simulink model "deltino"  (R2021b)
(part 4 of 10)

t2190 = t1608.*t2164;
t2191 = t1609.*t2165;
t2193 = t1606.*t2166;
t2194 = t1607.*t2167;
t2196 = t1632.*t2168;
t2197 = t1633.*t2169;
t2198 = t1630.*t2170;
t2199 = t1631.*t2171;
t2205 = -t2201;
t2206 = -t2202;
t2210 = -t2204;
t2211 = -t2207;
t2213 = -t2208;
t2214 = -t2209;
t2215 = -t2212;
t2216 = t1369+t1722+t1745+t2007;
t2217 = t1371+t1724+t1748+t2008;
t2218 = t1373+t1726+t1751+t2009;
t2219 = t1375+t1728+t1754+t2010;
t2220 = t1370+t1723+t1746+t2022;
t2221 = t1372+t1725+t1749+t2023;
t2222 = t1374+t1727+t1752+t2024;
t2223 = t1376+t1729+t1755+t2025;
t2224 = t1422+t1689+t1758+t2026;
t2225 = t1425+t1692+t1764+t2028;
t2226 = t1428+t1695+t1770+t2030;
t2227 = t1431+t1698+t1776+t2032;
t2228 = t1458+t1660+t1788+t2027;
t2229 = t1459+t1661+t1789+t2029;
t2230 = t1460+t1662+t1791+t2031;
t2231 = t1461+t1663+t1794+t2033;
t2232 = p2x_dot+t47+t454+t459+t472+t480+t482+t643+t699+t872+t893+t910+t1060+t1064+t1076+t1207+t1211+t1317+t1763;
t2233 = p1x_dot+t47+t442+t454+t459+t472+t482+t641+t790+t872+t932+t1048+t1058+t1060+t1064+t1206+t1210+t1314+t1757;
t2234 = p3x_dot+t47+t454+t459+t480+t645+t699+t767+t791+t872+t893+t910+t1060+t1064+t1076+t1208+t1212+t1320+t1769;
t2235 = t1871+t1975+t1996;
t2236 = p4x_dot+t47+t442+t454+t459+t647+t767+t790+t791+t872+t932+t1048+t1058+t1060+t1064+t1209+t1213+t1323+t1775;
t2237 = t1865+t1989+t1997;
t2238 = t1864+t1995+t2001;
t2241 = p2y_dot+t50+t477+t493+t700+t719+t726+t758+t761+t887+t909+t915+t922+t928+t1077+t1215+t1263+t1451+t1735;
t2242 = p3y_dot+t50+t449+t477+t700+t720+t758+t761+t800+t887+t909+t915+t922+t928+t1077+t1216+t1264+t1454+t1738;
t2243 = t1856+t2002+t2006;
t2246 = p1y_dot+t50+t457+t460+t477+t493+t700+t718+t726+t887+t909+t1061+t1067+t1073+t1077+t1214+t1262+t1450+t1732;
t2247 = p4y_dot+t50+t449+t457+t460+t477+t700+t721+t800+t887+t909+t1061+t1067+t1073+t1077+t1217+t1265+t1457+t1741;
t2272 = t1549.*t2248;
t2273 = t1550.*t2249;
t2274 = t1578.*t2252;
t2275 = t1548.*t2253;
t2276 = t1579.*t2256;
t2277 = t1547.*t2257;
t2278 = t1577.*t2258;
t2279 = t1576.*t2259;
t2323 = p2y_dot+t50+t477+t493+t700+t726+t758+t761+t887+t909+t915+t922+t928+t1077+t1453+t1704+t1737+t2067;
t2324 = p3y_dot+t50+t449+t477+t700+t758+t761+t800+t887+t909+t915+t922+t928+t1077+t1456+t1706+t1740+t2069;
t1944 = -t1937;
t1947 = -t1941;
t1966 = p3y+t48+t1949;
t2112 = p3x+t45+t2084;
t2113 = p3x+t45+t2085;
t2114 = p4x+t45+t2086;
t2115 = p4x+t45+t2087;
t2116 = -t2105;
t2117 = p1x+t45+t2088;
t2118 = p1x+t45+t2089;
t2119 = p2x+t45+t2090;
t2120 = p2x+t45+t2091;
t2123 = p3y+t48+t2093;
t2127 = by+t57+t2102;
t2128 = p2y+t48+t2103;
t2132 = by+t59+t2108;
t2134 = p3y+t48+t2111;
t2145 = -t1983.*(t1230-t1555);
t2147 = -t1985.*(t1232-t1557);
t2149 = t1828.*t1994;
t2150 = -t1990.*(t1226-t1551);
t2152 = -t1992.*(t1228-t1553);
t2154 = t1826.*t1999;
t2155 = t1827.*t2000;
t2156 = t1983.*(t1230-t1555);
t2157 = t1829.*t2004;
t2163 = -t2034.*(t1276-t1561);
t2176 = t1919.*t2047;
t2177 = -t2173;
t2178 = t1921.*t2049;
t2179 = t1923.*t2046;
t2180 = -t2175;
t2181 = t1924.*t2048;
t2182 = t1953.*t2016;
t2183 = t1954.*t2017;
t2184 = t1956.*t2014;
t2185 = t1957.*t2015;
t2186 = t1955.*t2018;
t2187 = t1958.*t2021;
t2188 = t1959.*t2019;
t2195 = -t2190;
t2200 = -t2197;
t2239 = 1.0./t2235;
t2244 = 1.0./t2237;
t2250 = 1.0./t2238;
t2254 = 1.0./t2243;
t2260 = t1515.*t2232;
t2261 = t1514.*t2233;
t2263 = t1516.*t2234;
t2265 = t1517.*t2236;
t2268 = -t2241.*(t404-(t7.*t1159)./5.0);
t2269 = -t2242.*(t405-(t10.*t1159)./5.0);
t2270 = -t2246.*(t403-(t4.*t1159)./5.0);
t2271 = -t2247.*(t406-(t13.*t1159)./5.0);
t2280 = t1929+t2109+t2121;
t2281 = t1927+t2110+t2130;
t2282 = t1930+t2106+t2126;
t2301 = t2122.*t2224;
t2306 = t2129.*t2227;
t2310 = t2131.*t2225;
t2315 = p2x_dot+t47+t454+t459+t472+t480+t482+t699+t872+t893+t910+t1060+t1064+t1076+t1318+t1718+t1765+t2073;
t2316 = bx_dot+t65+t472+t480+t482+t699+t755+t760+t893+t910+t914+t918+t1039+t1076+t1365+t1699+t1793+t2056;
t2317 = p1x_dot+t47+t442+t454+t459+t472+t482+t790+t872+t932+t1048+t1058+t1060+t1064+t1315+t1716+t1759+t2072;
t2318 = p2x_dot+t47+t454+t459+t472+t480+t482+t699+t872+t893+t910+t1060+t1064+t1076+t1319+t1719+t1767+t2075;
t2319 = bx_dot+t64+t442+t472+t482+t755+t760+t790+t914+t918+t932+t1039+t1048+t1058+t1363+t1696+t1790+t2055;
t2320 = bx_dot+t65+t472+t480+t482+t699+t755+t760+t893+t910+t914+t918+t1039+t1076+t1366+t1700+t1795+t2063;
t2321 = p1x_dot+t47+t442+t454+t459+t472+t482+t790+t872+t932+t1048+t1058+t1060+t1064+t1316+t1717+t1761+t2074;
t2322 = bx_dot+t64+t442+t472+t482+t755+t760+t790+t914+t918+t932+t1039+t1048+t1058+t1364+t1697+t1792+t2062;
t2325 = by_dot+t71+t443+t449+t758+t761+t788+t800+t915+t922+t928+t933+t1045+t1057+t1410+t1720+t1780+t2064;
t2326 = by_dot+t71+t443+t449+t758+t761+t788+t800+t915+t922+t928+t933+t1045+t1057+t1411+t1665+t1781+t2076;
t2327 = p2y_dot+t50+t477+t493+t700+t726+t758+t761+t887+t909+t915+t922+t928+t1077+t1452+t1703+t1736+t2077;
t2328 = p3y_dot+t50+t449+t477+t700+t758+t761+t800+t887+t909+t915+t922+t928+t1077+t1455+t1705+t1739+t2078;
t2329 = by_dot+t72+t443+t493+t726+t758+t761+t788+t915+t922+t928+t933+t1045+t1057+t1419+t1721+t1782+t2070;
t2330 = by_dot+t72+t443+t493+t726+t758+t761+t788+t915+t922+t928+t933+t1045+t1057+t1420+t1668+t1783+t2079;
t2336 = -1.0./(-t1932+t1985.*(t1232-t1557)+t2003.*(t1281-t1562));
t2337 = 1.0./(-t1932+t1985.*(t1232-t1557)+t2003.*(t1281-t1562)).^2;
t2343 = -1.0./(t1933+t1990.*(t1226-t1551)+t1998.*(t1266-t1559));
t2344 = 1.0./(t1933+t1990.*(t1226-t1551)+t1998.*(t1266-t1559)).^2;
t2351 = -1.0./(t1931+t1992.*(t1228-t1553)+t2011.*(t1271-t1560));
t2352 = 1.0./(t1931+t1992.*(t1228-t1553)+t2011.*(t1271-t1560)).^2;
t2364 = t1889.*t2323;
t2365 = t1890.*t2324;
t2380 = (t2165.*-2.0e+2)./(-t1932+t1985.*(t1232-t1557)+t2003.*(t1281-t1562));
t2381 = (t2165.*2.0e+2)./(-t1932+t1985.*(t1232-t1557)+t2003.*(t1281-t1562));
t2383 = (t2166.*-2.0e+2)./(t1933+t1990.*(t1226-t1551)+t1998.*(t1266-t1559));
t2386 = (t2166.*2.0e+2)./(t1933+t1990.*(t1226-t1551)+t1998.*(t1266-t1559));
t2387 = (t2167.*-2.0e+2)./(t1931+t1992.*(t1228-t1553)+t2011.*(t1271-t1560));
t2392 = (t2167.*2.0e+2)./(t1931+t1992.*(t1228-t1553)+t2011.*(t1271-t1560));
t2436 = t2036+t2124+t2203+t2205+t2272+t2274;
t2437 = t2038+t2125+t2206+t2210+t2273+t2276;
t2438 = t2037+t2136+t2214+t2215+t2275+t2278;
t2439 = t2039+t2135+t2211+t2213+t2277+t2279;
t2133 = -t1966.*(t405-(t10.*t1159)./5.0);
t2160 = -t2157;
t2189 = t1966.*t2020;
t2240 = t2239.^2;
t2245 = t2244.^2;
t2251 = t2250.^2;
t2255 = t2254.^2;
t2262 = -t2260;
t2264 = -t2261;
t2266 = -t2263;
t2267 = -t2265;
t2284 = 1.0./t2280;
t2286 = 1.0./t2281;
t2288 = 1.0./t2282;
t2290 = -1.0./(t2105+t1853.*(t211./5.0-t248)+t1966.*(t405-(t10.*t1159)./5.0));
t2291 = 1.0./(t2105+t1853.*(t211./5.0-t248)+t1966.*(t405-(t10.*t1159)./5.0)).^2;
t2292 = t2112.*t2218;
t2293 = t2114.*t2219;
t2294 = t2117.*t2216;
t2295 = t2119.*t2217;
t2296 = t2113.*t2222;
t2297 = t2115.*t2223;
t2298 = t2118.*t2220;
t2299 = t2120.*t2221;
t2305 = t2123.*t2230;
t2309 = t2127.*t2228;
t2311 = t2128.*t2229;
t2312 = t2134.*t2226;
t2313 = t2132.*t2231;
t2331 = t1932+t2147+t2161;
t2332 = t1947+t2146+t2149;
t2333 = t1936+t2150+t2159;
t2334 = t1944+t2153+t2155;
t2338 = t1940+t2154+t2158;
t2339 = t1935+t2152+t2162;
t2340 = t1934+t2156+t2163;
t2341 = -1.0./(t1941-t2149+t1984.*(t1231-t1556));
t2342 = 1.0./(t1941-t2149+t1984.*(t1231-t1556)).^2;
t2345 = -1.0./(t1937-t2155+t1993.*(t1229-t1554));
t2346 = 1.0./(t1937-t2155+t1993.*(t1229-t1554)).^2;
t2347 = -1.0./(-t1938+t2157+t1986.*(t1233-t1558));
t2348 = 1.0./(-t1938+t2157+t1986.*(t1233-t1558)).^2;
t2355 = t2315.*(t1679-(t8.*t1070)./5.0);
t2356 = t2316.*(t1683-(t14.*t1070)./5.0);
t2357 = t2317.*(t1677-(t5.*t1070)./5.0);
t2358 = t2318.*(t1680-(t9.*t1070)./5.0);
t2359 = t2319.*(t1681-(t11.*t1070)./5.0);
t2360 = t2320.*(t1684-(t15.*t1070)./5.0);
t2361 = t2321.*(t1678-(t6.*t1070)./5.0);
t2362 = t2322.*(t1682-(t12.*t1070)./5.0);
t2367 = t1888.*t2326;
t2368 = t1891.*t2330;
t2369 = t2325.*(t1685-(t5.*t1159)./5.0);
t2371 = t2327.*(t1686-(t8.*t1159)./5.0);
t2372 = t2328.*(t1687-(t11.*t1159)./5.0);
t2373 = t2329.*(t1688-(t14.*t1159)./5.0);
t2379 = t2080./(t2105+t1853.*(t211./5.0-t248)+t1966.*(t405-(t10.*t1159)./5.0));
t2382 = (t2168.*-2.0e+2)./(t1941-t2149+t1984.*(t1231-t1556));
t2384 = (t2168.*2.0e+2)./(t1941-t2149+t1984.*(t1231-t1556));
t2385 = (t2169.*-2.0e+2)./(-t1938+t2157+t1986.*(t1233-t1558));
t2388 = (t2171.*-2.0e+2)./(t1937-t2155+t1993.*(t1229-t1554));
t2390 = (t2169.*2.0e+2)./(-t1938+t2157+t1986.*(t1233-t1558));
t2393 = (t2171.*2.0e+2)./(t1937-t2155+t1993.*(t1229-t1554));
t2408 = (t2316.*-2.0e+2)./(-t1932+t1985.*(t1232-t1557)+t2003.*(t1281-t1562));
t2409 = (t2316.*2.0e+2)./(-t1932+t1985.*(t1232-t1557)+t2003.*(t1281-t1562));
t2410 = (t2324.*-2.0e+2)./(t1941-t2149+t1984.*(t1231-t1556));
t2411 = (t2329.*-2.0e+2)./(-t1932+t1985.*(t1232-t1557)+t2003.*(t1281-t1562));
t2412 = (t2317.*-2.0e+2)./(t1933+t1990.*(t1226-t1551)+t1998.*(t1266-t1559));
t2413 = (t2315.*-2.0e+2)./(t1931+t1992.*(t1228-t1553)+t2011.*(t1271-t1560));
t2414 = (t2318.*-2.0e+2)./(t1937-t2155+t1993.*(t1229-t1554));
t2415 = (t2322.*-2.0e+2)./(t1941-t2149+t1984.*(t1231-t1556));
t2416 = (t2320.*-2.0e+2)./(-t1938+t2157+t1986.*(t1233-t1558));
t2417 = (t2323.*-2.0e+2)./(t1937-t2155+t1993.*(t1229-t1554));
t2418 = (t2329.*2.0e+2)./(-t1932+t1985.*(t1232-t1557)+t2003.*(t1281-t1562));
t2419 = (t2322.*2.0e+2)./(t1941-t2149+t1984.*(t1231-t1556));
t2420 = (t2320.*2.0e+2)./(-t1938+t2157+t1986.*(t1233-t1558));
t2423 = (t2325.*-2.0e+2)./(t1933+t1990.*(t1226-t1551)+t1998.*(t1266-t1559));
t2424 = (t2330.*-2.0e+2)./(-t1938+t2157+t1986.*(t1233-t1558));
t2426 = (t2325.*2.0e+2)./(t1933+t1990.*(t1226-t1551)+t1998.*(t1266-t1559));
t2428 = (t2327.*-2.0e+2)./(t1931+t1992.*(t1228-t1553)+t2011.*(t1271-t1560));
t2429 = (t2330.*2.0e+2)./(-t1938+t2157+t1986.*(t1233-t1558));
t2192 = -t2189;
t2283 = t1926+t2116+t2133;
t2285 = t2284.^2;
t2287 = t2286.^2;
t2289 = t2288.^2;
t2300 = -t2293;
t2302 = -t2294;
t2303 = -t2295;
t2304 = -t2296;
t2307 = -t2298;
t2308 = -t2299;
t2314 = -t2309;
t2335 = t1938+t2148+t2160;
t2349 = 1.0./t2338;
t2353 = 1.0./t2340;
t2363 = -t2356;
t2366 = -t2362;
t2370 = -t2367;
t2374 = -t2371;
t2375 = t2082.*t2284;
t2376 = t2081.*t2288;
t2377 = t2083.*t2286;
t2378 = t2080.*t2290;
t2394 = t2233.*t2284;
t2395 = t2232.*t2286;
t2398 = t2234.*t2290;
t2399 = t2236.*t2288;
t2401 = t2246.*t2284;
t2402 = t2241.*t2286;
t2403 = t2242.*t2290;
t2404 = t2247.*t2288;
t2432 = t2050+t2144+t2185+t2188+t2262+t2268;
t2433 = t2051+t2143+t2184+t2186+t2264+t2270;
t2434 = t2057+t2142+t2183+t2187+t2267+t2271;
t2465 = t2180+t2195+t2292+t2312+t2359+t2372;
t2467 = t2178+t2200+t2297+t2313+t2360+t2368;
t2481 = t1916.*t2337.*(t2173-t2191+t2293-t2306+t2356-t2373).*-4.0e+4;
t2495 = t2114.*t2337.*(t2173-t2191+t2293-t2306+t2356-t2373).*-4.0e+4;
t2496 = t2114.*t2337.*(t2173-t2191+t2293-t2306+t2356-t2373).*4.0e+4;
t2498 = t2129.*t2337.*(t2173-t2191+t2293-t2306+t2356-t2373).*-4.0e+4;
t2350 = t2349.^2;
t2354 = t2353.^2;
t2389 = t2164.*t2353.*2.0e+2;
t2391 = t2170.*t2349.*2.0e+2;
t2396 = -t2394;
t2397 = -t2395;
t2400 = -t2399;
t2405 = -t2401;
t2406 = -t2402;
t2407 = -t2404;
t2421 = t2321.*t2349.*2.0e+2;
t2422 = t2319.*t2353.*2.0e+2;
t2427 = t2326.*t2349.*2.0e+2;
t2430 = t2328.*t2353.*2.0e+2;
t2435 = t2052+t2141+t2182+t2192+t2266+t2269;
t2440 = t1848.*t2287.*t2432;
t2441 = t1852.*t2285.*t2433;
t2444 = t1861.*t2289.*t2434;
t2448 = t1955.*t2285.*t2433;
t2449 = t1956.*t2285.*t2433;
t2450 = t1957.*t2287.*t2432;
t2451 = t1959.*t2287.*t2432;
t2454 = t1954.*t2289.*t2434;
t2455 = t1958.*t2289.*t2434;
t2461 = t2174+t2193+t2301+t2302+t2357+t2369;
t2462 = t2177+t2191+t2300+t2306+t2363+t2373;
t2463 = t2172+t2194+t2303+t2310+t2355+t2374;
t2464 = t2176+t2199+t2308+t2311+t2358+t2364;
t2466 = t2181+t2196+t2304+t2305+t2365+t2366;
t2468 = t2179+t2198+t2307+t2314+t2361+t2370;
t2489 = t1921.*t2348.*t2467.*4.0e+4;
t2504 = t2115.*t2348.*t2467.*4.0e+4;
t2514 = t2132.*t2348.*t2467.*4.0e+4;
t2520 = t2381+t2481;
t2528 = t2409+t2496;
t2530 = t2418+t2498;
t2425 = -t2421;
t2431 = -t2430;
t2442 = -t2440;
t2443 = -t2441;
t2445 = t1853.*t2291.*t2435;
t2446 = -t2444;
t2447 = (t1853.*t2290.*t2435)./(t2105+t1853.*(t211./5.0-t248)+t1966.*(t405-(t10.*t1159)./5.0));
t2452 = -t2449;
t2453 = -t2450;
t2456 = t1953.*t2291.*t2435;
t2457 = -t2454;
t2458 = (t1953.*t2290.*t2435)./(t2105+t1853.*(t211./5.0-t248)+t1966.*(t405-(t10.*t1159)./5.0));
t2459 = t1966.*t2291.*t2435;
t2460 = (t1966.*t2290.*t2435)./(t2105+t1853.*(t211./5.0-t248)+t1966.*(t405-(t10.*t1159)./5.0));
t2475 = t2405+t2448;
t2476 = t2406+t2451;
t2479 = t2407+t2455;
t2482 = t1918.*t2344.*t2461.*4.0e+4;
t2484 = t1915.*t2352.*t2463.*4.0e+4;
t2485 = t1919.*t2346.*t2464.*4.0e+4;
t2488 = t1924.*t2342.*t2466.*4.0e+4;
t2491 = -t2489;
t2492 = t1920.*t2354.*t2465.*4.0e+4;
t2493 = t1923.*t2350.*t2468.*4.0e+4;
t2497 = t2117.*t2344.*t2461.*4.0e+4;
t2500 = t2113.*t2342.*t2466.*4.0e+4;
t2501 = t2122.*t2344.*t2461.*4.0e+4;
t2502 = t2120.*t2346.*t2464.*4.0e+4;
t2505 = t2119.*t2352.*t2463.*4.0e+4;
t2507 = t2123.*t2342.*t2466.*4.0e+4;
t2509 = t2112.*t2354.*t2465.*4.0e+4;
t2510 = t2128.*t2346.*t2464.*4.0e+4;
t2513 = t2131.*t2352.*t2463.*4.0e+4;
t2515 = -t2514;
t2516 = t2134.*t2354.*t2465.*4.0e+4;
t2517 = t2118.*t2350.*t2468.*4.0e+4;
t2519 = t2127.*t2350.*t2468.*4.0e+4;
S_dot = ft_5({bx,bx_dot,by,by_dot,p1x,p1x_dot,p1y,p1y_dot,p2x,p2x_dot,p2y,p2y_dot,p4x,p4x_dot,p4y,p4y_dot,phi_dot,psi_dot,t10,t1006,t1012,t1013,t1014,t1015,t1016,t1018,t102,t1027,t1028,t1030,t1031,t1033,t1037,t1039,t1040,t1045,t1046,t1047,t1048,t1049,t1051,t1052,t1053,t1054,t1056,t1057,t1058,t1059,t1060,t1061,t1062,t1063,t1064,t1065,t1066,t1067,t1069,t1070,t1071,t1072,t1073,t1074,t1075,t1076,t1077,t1078,t1079,t1081,t1083,t1084,t1086,t1087,t1089,t1091,t1092,t1093,t1094,t1096,t1098,t11,t1105,t1106,t1108,t1109,t1111,t1115,t1126,t1127,t1129,t1131,t1133,t1134,t1135,t1136,t1138,t1139,t1150,t1151,t1159,t1160,t1165,t1171,t1172,t12,t1208,t1212,t1216,t1226,t1228,t1229,t1231,t1232,t1233,t1264,t1266,t1271,t1281,t13,t1315,t1316,t1318,t1319,t1320,t1326,t1365,t1366,t1367,t1393,t14,t1408,t1410,t1411,t1436,t144,t145,t1452,t1453,t1454,t1455,t1456,t146,t147,t148,t149,t15,t150,t151,t152,t153,t1533,t1534,t154,t155,t1551,t1553,t1554,t1556,t1557,t1558,t1559,t1560,t1562,t1564,t1570,t1571,t1572,t1582,t1583,t1599,t16,t1600,t1601,t161,t1610,t1611,t1614,t162,t1629,t163,t1634,t1635,t1636,t1637,t164,t1642,t1643,t1644,t1645,t165,t166,t1664,t1665,t1699,t17,t1700,t1701,t1703,t1704,t1705,t1706,t1707,t1716,t1717,t1718,t1719,t1720,t1730,t1731,t1736,t1737,t1738,t1739,t1740,t1742,t1743,t175,t1759,t176,t1761,t1765,t1767,t1769,t177,t1771,t1773,t1780,t1781,t1793,t1795,t1796,t18,t180,t1809,t181,t1810,t1823,t183,t1847,t1851,t1853,t1858,t1859,t1860,t1866,t1867,t1868,t187,t1872,t1873,t1874,t1875,t1876,t1877,t1878,t1879,t1896,t1897,t1898,t1899,t19,t190,t1900,t1901,t1902,t1903,t1904,t1905,t1906,t1907,t1915,t1916,t1918,t1919,t1920,t1921,t1923,t1924,t1931,t1932,t1933,t1937,t1938,t1939,t1941,t1942,t1943,t1945,t1946,t1948,t1949,t1950,t1951,t1952,t1953,t1960,t1961,t1962,t1963,t1964,t1965,t1966,t1967,t1968,t1969,t1970,t1971,t1972,t1973,t1974,t1984,t1985,t1986,t1990,t1992,t1993,t1998,t2,t20,t2003,t2005,t2011,t2012,t2013,t2035,t2044,t2045,t2055,t2056,t2058,t2059,t2062,t2063,t2064,t2067,t2069,t207,t2070,t2071,t2072,t2073,t2074,t2075,t2076,t2077,t2078,t208,t2084,t2085,t2086,t2087,t2088,t2089,t209,t2090,t2091,t2092,t2093,t21,t210,t2102,t2103,t2104,t2105,t2107,t2108,t211,t2111,t2112,t2113,t2114,t2115,t2117,t2118,t2119,t212,t2120,t2122,t2123,t2127,t2128,t2129,t2131,t2132,t2134,t214,t2149,t2155,t2157,t2164,t2165,t2166,t2167,t2168,t2169,t217,t2170,t2171,t2173,t218,t219,t2191,t22,t2201,t2202,t2203,t2204,t2207,t2208,t2209,t221,t2212,t222,t223,t2234,t2239,t2240,t2242,t2244,t2245,t2248,t2249,t225,t2250,t2251,t2252,t2253,t2254,t2255,t2256,t2257,t2258,t2259,t2272,t2273,t2274,t2275,t2276,t2277,t2278,t2279,t2290,t2293,t23,t2306,t2315,t2316,t2317,t2318,t2319,t2320,t2321,t2322,t2323,t2324,t2325,t2326,t2327,t2328,t2329,t233,t2330,t2337,t2342,t2344,t2346,t2348,t2349,t2350,t2352,t2353,t2354,t2356,t236,t237,t2373,t2375,t2376,t2377,t2379,t238,t2384,t2386,t2389,t2390,t2391,t2392,t2393,t2396,t2397,t2398,t24,t2400,t2403,t241,t2410,t2412,t2413,t2414,t2417,t2419,t242,t2420,t2422,t2425,t2426,t2427,t2428,t2429,t243,t2431,t2435,t244,t2442,t2443,t2446,t2447,t245,t2452,t2453,t2457,t2458,t246,t2460,t2461,t2463,t2464,t2465,t2466,t2467,t2468,t247,t2475,t2476,t2479,t248,t2482,t2484,t2485,t2488,t249,t2491,t2492,t2493,t2497,t25,t2500,t2501,t2502,t2504,t2505,t2507,t2509,t2510,t2513,t2515,t2516,t2517,t2519,t252,t2520,t2528,t2530,t254,t255,t256,t257,t258,t26,t260,t261,t265,t267,t27,t270,t272,t273,t28,t29,t3,t30,t308,t31,t312,t316,t317,t318,t319,t322,t324,t328,t329,t341,t343,t350,t351,t352,t353,t354,t358,t359,t360,t361,t362,t366,t367,t368,t369,t371,t374,t375,t376,t377,t379,t380,t381,t383,t4,t402,t403,t404,t405,t406,t419,t420,t422,t423,t424,t427,t429,t431,t437,t442,t443,t444,t445,t446,t449,t450,t454,t455,t456,t457,t458,t459,t460,t461,t462,t464,t465,t470,t471,t472,t474,t475,t477,t478,t479,t480,t481,t482,t483,t485,t486,t488,t489,t490,t492,t493,t494,t5,t501,t502,t504,t529,t530,t531,t532,t533,t535,t536,t539,t540,t541,t542,t543,t544,t545,t548,t549,t552,t558,t561,t562,t563,t570,t572,t577,t578,t580,t6,t601,t603,t607,t609,t610,t612,t614,t620,t641,t643,t645,t647,t661,t663,t667,t669,t670,t672,t673,t674,t676,t678,t680,t684,t698,t699,t7,t700,t701,t718,t719,t720,t721,t722,t723,t725,t726,t728,t731,t733,t737,t754,t755,t756,t757,t758,t759,t760,t761,t762,t763,t765,t767,t768,t77,t770,t771,t777,t778,t78,t780,t781,t783,t784,t786,t787,t788,t789,t79,t790,t791,t792,t794,t795,t796,t797,t798,t799,t8,t80,t800,t801,t802,t804,t805,t806,t807,t808,t809,t81,t814,t815,t816,t817,t82,t825,t827,t831,t836,t837,t84,t840,t845,t846,t847,t848,t85,t851,t86,t87,t872,t873,t88,t882,t885,t887,t888,t889,t89,t890,t891,t892,t893,t894,t896,t9,t90,t907,t908,t909,t91,t910,t911,t913,t914,t915,t916,t917,t918,t919,t92,t920,t921,t922,t924,t925,t926,t927,t928,t93,t930,t932,t933,t934,t935,t936,t94,t945,t947,t949,t95,t951,t953,t954,t955,t957,t959,t961,t963,t964,t966,t967,t972,t981,t982,t984,t985,t987,t991,t993,t995,t999,th11_dot,th12_dot,th13_dot,th21_dot,th22_dot,th23_dot,th31_dot,th32_dot,th33_dot,th41_dot,th42_dot,th43_dot,zeta_dot});
end
function S_dot = ft_5(ct)
bx = ct{1};
bx_dot = ct{2};
by = ct{3};
by_dot = ct{4};
p1x = ct{5};
p1x_dot = ct{6};
p1y = ct{7};
p1y_dot = ct{8};
p2x = ct{9};
p2x_dot = ct{10};
p2y = ct{11};
p2y_dot = ct{12};
p4x = ct{13};
p4x_dot = ct{14};
p4y = ct{15};
p4y_dot = ct{16};
phi_dot = ct{17};
psi_dot = ct{18};
t10 = ct{19};
t1006 = ct{20};
t1012 = ct{21};
t1013 = ct{22};
t1014 = ct{23};
t1015 = ct{24};
t1016 = ct{25};
t1018 = ct{26};
t102 = ct{27};
t1027 = ct{28};
t1028 = ct{29};
t1030 = ct{30};
t1031 = ct{31};
t1033 = ct{32};
t1037 = ct{33};
t1039 = ct{34};
t1040 = ct{35};
t1045 = ct{36};
t1046 = ct{37};
t1047 = ct{38};
t1048 = ct{39};
t1049 = ct{40};
t1051 = ct{41};
t1052 = ct{42};
t1053 = ct{43};
t1054 = ct{44};
t1056 = ct{45};
t1057 = ct{46};
t1058 = ct{47};
t1059 = ct{48};
t1060 = ct{49};
t1061 = ct{50};
t1062 = ct{51};
t1063 = ct{52};
t1064 = ct{53};
t1065 = ct{54};
t1066 = ct{55};
t1067 = ct{56};
t1069 = ct{57};
t1070 = ct{58};
t1071 = ct{59};
t1072 = ct{60};
t1073 = ct{61};
t1074 = ct{62};
t1075 = ct{63};
t1076 = ct{64};
t1077 = ct{65};
t1078 = ct{66};
t1079 = ct{67};
t1081 = ct{68};
t1083 = ct{69};
t1084 = ct{70};
t1086 = ct{71};
t1087 = ct{72};
t1089 = ct{73};
t1091 = ct{74};
t1092 = ct{75};
t1093 = ct{76};
t1094 = ct{77};
t1096 = ct{78};
t1098 = ct{79};
t11 = ct{80};
t1105 = ct{81};
t1106 = ct{82};
t1108 = ct{83};
t1109 = ct{84};
t1111 = ct{85};
t1115 = ct{86};
t1126 = ct{87};
t1127 = ct{88};
t1129 = ct{89};
t1131 = ct{90};
t1133 = ct{91};
t1134 = ct{92};
t1135 = ct{93};
t1136 = ct{94};
t1138 = ct{95};
t1139 = ct{96};
t1150 = ct{97};
t1151 = ct{98};
t1159 = ct{99};
t1160 = ct{100};
t1165 = ct{101};
t1171 = ct{102};
t1172 = ct{103};
t12 = ct{104};
t1208 = ct{105};
t1212 = ct{106};
t1216 = ct{107};
t1226 = ct{108};
t1228 = ct{109};
t1229 = ct{110};
t1231 = ct{111};
t1232 = ct{112};
t1233 = ct{113};
t1264 = ct{114};
t1266 = ct{115};
t1271 = ct{116};
t1281 = ct{117};
t13 = ct{118};
t1315 = ct{119};
t1316 = ct{120};
t1318 = ct{121};
t1319 = ct{122};
t1320 = ct{123};
t1326 = ct{124};
t1365 = ct{125};
t1366 = ct{126};
t1367 = ct{127};
t1393 = ct{128};
t14 = ct{129};
t1408 = ct{130};
t1410 = ct{131};
t1411 = ct{132};
t1436 = ct{133};
t144 = ct{134};
t145 = ct{135};
t1452 = ct{136};
t1453 = ct{137};
t1454 = ct{138};
t1455 = ct{139};
t1456 = ct{140};
t146 = ct{141};
t147 = ct{142};
t148 = ct{143};
t149 = ct{144};
t15 = ct{145};
t150 = ct{146};
t151 = ct{147};
t152 = ct{148};
t153 = ct{149};
t1533 = ct{150};
t1534 = ct{151};
t154 = ct{152};
t155 = ct{153};
t1551 = ct{154};
t1553 = ct{155};
t1554 = ct{156};
t1556 = ct{157};
t1557 = ct{158};
t1558 = ct{159};
t1559 = ct{160};
t1560 = ct{161};
t1562 = ct{162};
t1564 = ct{163};
t1570 = ct{164};
t1571 = ct{165};
t1572 = ct{166};
t1582 = ct{167};
t1583 = ct{168};
t1599 = ct{169};
t16 = ct{170};
t1600 = ct{171};
t1601 = ct{172};
t161 = ct{173};
t1610 = ct{174};
t1611 = ct{175};
t1614 = ct{176};
t162 = ct{177};
t1629 = ct{178};
t163 = ct{179};
t1634 = ct{180};
t1635 = ct{181};
t1636 = ct{182};
t1637 = ct{183};
t164 = ct{184};
t1642 = ct{185};
t1643 = ct{186};
t1644 = ct{187};
t1645 = ct{188};
t165 = ct{189};
t166 = ct{190};
t1664 = ct{191};
t1665 = ct{192};
t1699 = ct{193};
t17 = ct{194};
t1700 = ct{195};
t1701 = ct{196};
t1703 = ct{197};
t1704 = ct{198};
t1705 = ct{199};
t1706 = ct{200};
t1707 = ct{201};
t1716 = ct{202};
t1717 = ct{203};
t1718 = ct{204};
t1719 = ct{205};
t1720 = ct{206};
t1730 = ct{207};
t1731 = ct{208};
t1736 = ct{209};
t1737 = ct{210};
t1738 = ct{211};
t1739 = ct{212};
t1740 = ct{213};
t1742 = ct{214};
t1743 = ct{215};
t175 = ct{216};
t1759 = ct{217};
t176 = ct{218};
t1761 = ct{219};
t1765 = ct{220};
t1767 = ct{221};
t1769 = ct{222};
t177 = ct{223};
t1771 = ct{224};
t1773 = ct{225};
t1780 = ct{226};
t1781 = ct{227};
t1793 = ct{228};
t1795 = ct{229};
t1796 = ct{230};
t18 = ct{231};
t180 = ct{232};
t1809 = ct{233};
t181 = ct{234};
t1810 = ct{235};
t1823 = ct{236};
t183 = ct{237};
t1847 = ct{238};
t1851 = ct{239};
t1853 = ct{240};
t1858 = ct{241};
t1859 = ct{242};
t1860 = ct{243};
t1866 = ct{244};
t1867 = ct{245};
t1868 = ct{246};
t187 = ct{247};
t1872 = ct{248};
t1873 = ct{249};
t1874 = ct{250};
t1875 = ct{251};
t1876 = ct{252};
t1877 = ct{253};
t1878 = ct{254};
t1879 = ct{255};
t1896 = ct{256};
t1897 = ct{257};
t1898 = ct{258};
t1899 = ct{259};
t19 = ct{260};
t190 = ct{261};
t1900 = ct{262};
t1901 = ct{263};
t1902 = ct{264};
t1903 = ct{265};
t1904 = ct{266};
t1905 = ct{267};
t1906 = ct{268};
t1907 = ct{269};
t1915 = ct{270};
t1916 = ct{271};
t1918 = ct{272};
t1919 = ct{273};
t1920 = ct{274};
t1921 = ct{275};
t1923 = ct{276};
t1924 = ct{277};
t1931 = ct{278};
t1932 = ct{279};
t1933 = ct{280};
t1937 = ct{281};
t1938 = ct{282};
t1939 = ct{283};
t1941 = ct{284};
t1942 = ct{285};
t1943 = ct{286};
t1945 = ct{287};
t1946 = ct{288};
t1948 = ct{289};
t1949 = ct{290};
t1950 = ct{291};
t1951 = ct{292};
t1952 = ct{293};
t1953 = ct{294};
t1960 = ct{295};
t1961 = ct{296};
t1962 = ct{297};
t1963 = ct{298};
t1964 = ct{299};
t1965 = ct{300};
t1966 = ct{301};
t1967 = ct{302};
t1968 = ct{303};
t1969 = ct{304};
t1970 = ct{305};
t1971 = ct{306};
t1972 = ct{307};
t1973 = ct{308};
t1974 = ct{309};
t1984 = ct{310};
t1985 = ct{311};
t1986 = ct{312};
t1990 = ct{313};
t1992 = ct{314};
t1993 = ct{315};
t1998 = ct{316};
t2 = ct{317};
t20 = ct{318};
t2003 = ct{319};
t2005 = ct{320};
t2011 = ct{321};
t2012 = ct{322};
t2013 = ct{323};
t2035 = ct{324};
t2044 = ct{325};
t2045 = ct{326};
t2055 = ct{327};
t2056 = ct{328};
t2058 = ct{329};
t2059 = ct{330};
t2062 = ct{331};
t2063 = ct{332};
t2064 = ct{333};
t2067 = ct{334};
t2069 = ct{335};
t207 = ct{336};
t2070 = ct{337};
t2071 = ct{338};
t2072 = ct{339};
t2073 = ct{340};
t2074 = ct{341};
t2075 = ct{342};
t2076 = ct{343};
t2077 = ct{344};
t2078 = ct{345};
t208 = ct{346};
t2084 = ct{347};
t2085 = ct{348};
t2086 = ct{349};
t2087 = ct{350};
t2088 = ct{351};
t2089 = ct{352};
t209 = ct{353};
t2090 = ct{354};
t2091 = ct{355};
t2092 = ct{356};
t2093 = ct{357};
t21 = ct{358};
t210 = ct{359};
t2102 = ct{360};
t2103 = ct{361};
t2104 = ct{362};
t2105 = ct{363};
t2107 = ct{364};
t2108 = ct{365};
t211 = ct{366};
t2111 = ct{367};
t2112 = ct{368};
t2113 = ct{369};
t2114 = ct{370};
t2115 = ct{371};
t2117 = ct{372};
t2118 = ct{373};
t2119 = ct{374};
t212 = ct{375};
t2120 = ct{376};
t2122 = ct{377};
t2123 = ct{378};
t2127 = ct{379};
t2128 = ct{380};
t2129 = ct{381};
t2131 = ct{382};
t2132 = ct{383};
t2134 = ct{384};
t214 = ct{385};
t2149 = ct{386};
t2155 = ct{387};
t2157 = ct{388};
t2164 = ct{389};
t2165 = ct{390};
t2166 = ct{391};
t2167 = ct{392};
t2168 = ct{393};
t2169 = ct{394};
t217 = ct{395};
t2170 = ct{396};
t2171 = ct{397};
t2173 = ct{398};
t218 = ct{399};
t219 = ct{400};
t2191 = ct{401};
t22 = ct{402};
t2201 = ct{403};
t2202 = ct{404};
t2203 = ct{405};
t2204 = ct{406};
t2207 = ct{407};
t2208 = ct{408};
t2209 = ct{409};
t221 = ct{410};
t2212 = ct{411};
t222 = ct{412};
t223 = ct{413};
t2234 = ct{414};
t2239 = ct{415};
t2240 = ct{416};
t2242 = ct{417};
t2244 = ct{418};
t2245 = ct{419};
t2248 = ct{420};
t2249 = ct{421};
t225 = ct{422};
t2250 = ct{423};
t2251 = ct{424};
t2252 = ct{425};
t2253 = ct{426};
t2254 = ct{427};
t2255 = ct{428};
t2256 = ct{429};
t2257 = ct{430};
t2258 = ct{431};
t2259 = ct{432};
t2272 = ct{433};
t2273 = ct{434};
t2274 = ct{435};
t2275 = ct{436};
t2276 = ct{437};
t2277 = ct{438};
t2278 = ct{439};
t2279 = ct{440};
t2290 = ct{441};
t2293 = ct{442};
t23 = ct{443};
t2306 = ct{444};
t2315 = ct{445};
t2316 = ct{446};
t2317 = ct{447};
t2318 = ct{448};
t2319 = ct{449};
t2320 = ct{450};
t2321 = ct{451};
t2322 = ct{452};
t2323 = ct{453};
t2324 = ct{454};
t2325 = ct{455};
t2326 = ct{456};
t2327 = ct{457};
t2328 = ct{458};
t2329 = ct{459};
t233 = ct{460};
t2330 = ct{461};
t2337 = ct{462};
t2342 = ct{463};
t2344 = ct{464};
t2346 = ct{465};
t2348 = ct{466};
t2349 = ct{467};
t2350 = ct{468};
t2352 = ct{469};
t2353 = ct{470};
t2354 = ct{471};
t2356 = ct{472};
t236 = ct{473};
t237 = ct{474};
t2373 = ct{475};
t2375 = ct{476};
t2376 = ct{477};
t2377 = ct{478};
t2379 = ct{479};
t238 = ct{480};
t2384 = ct{481};
t2386 = ct{482};
t2389 = ct{483};
t2390 = ct{484};
t2391 = ct{485};
t2392 = ct{486};
t2393 = ct{487};
t2396 = ct{488};
t2397 = ct{489};
t2398 = ct{490};
t24 = ct{491};
t2400 = ct{492};
t2403 = ct{493};
t241 = ct{494};
t2410 = ct{495};
t2412 = ct{496};
t2413 = ct{497};
t2414 = ct{498};
t2417 = ct{499};
t2419 = ct{500};
t242 = ct{501};
t2420 = ct{502};
t2422 = ct{503};
t2425 = ct{504};
t2426 = ct{505};
t2427 = ct{506};
t2428 = ct{507};
t2429 = ct{508};
t243 = ct{509};
t2431 = ct{510};
t2435 = ct{511};
t244 = ct{512};
t2442 = ct{513};
t2443 = ct{514};
t2446 = ct{515};
t2447 = ct{516};
t245 = ct{517};
t2452 = ct{518};
t2453 = ct{519};
t2457 = ct{520};
t2458 = ct{521};
t246 = ct{522};
t2460 = ct{523};
t2461 = ct{524};
t2463 = ct{525};
t2464 = ct{526};
t2465 = ct{527};
t2466 = ct{528};
t2467 = ct{529};
t2468 = ct{530};
t247 = ct{531};
t2475 = ct{532};
t2476 = ct{533};
t2479 = ct{534};
t248 = ct{535};
t2482 = ct{536};
t2484 = ct{537};
t2485 = ct{538};
t2488 = ct{539};
t249 = ct{540};
t2491 = ct{541};
t2492 = ct{542};
t2493 = ct{543};
t2497 = ct{544};
t25 = ct{545};
t2500 = ct{546};
t2501 = ct{547};
t2502 = ct{548};
t2504 = ct{549};
t2505 = ct{550};
t2507 = ct{551};
t2509 = ct{552};
t2510 = ct{553};
t2513 = ct{554};
t2515 = ct{555};
t2516 = ct{556};
t2517 = ct{557};
t2519 = ct{558};
t252 = ct{559};
t2520 = ct{560};
t2528 = ct{561};
t2530 = ct{562};
t254 = ct{563};
t255 = ct{564};
t256 = ct{565};
t257 = ct{566};
t258 = ct{567};
t26 = ct{568};
t260 = ct{569};
t261 = ct{570};
t265 = ct{571};
t267 = ct{572};
t27 = ct{573};
t270 = ct{574};
t272 = ct{575};
t273 = ct{576};
t28 = ct{577};
t29 = ct{578};
t3 = ct{579};
t30 = ct{580};
t308 = ct{581};
t31 = ct{582};
t312 = ct{583};
t316 = ct{584};
t317 = ct{585};
t318 = ct{586};
t319 = ct{587};
t322 = ct{588};
t324 = ct{589};
t328 = ct{590};
t329 = ct{591};
t341 = ct{592};
t343 = ct{593};
t350 = ct{594};
t351 = ct{595};
t352 = ct{596};
t353 = ct{597};
t354 = ct{598};
t358 = ct{599};
t359 = ct{600};
t360 = ct{601};
t361 = ct{602};
t362 = ct{603};
t366 = ct{604};
t367 = ct{605};
t368 = ct{606};
t369 = ct{607};
t371 = ct{608};
t374 = ct{609};
t375 = ct{610};
t376 = ct{611};
t377 = ct{612};
t379 = ct{613};
t380 = ct{614};
t381 = ct{615};
t383 = ct{616};
t4 = ct{617};
t402 = ct{618};
t403 = ct{619};
t404 = ct{620};
t405 = ct{621};
t406 = ct{622};
t419 = ct{623};
t420 = ct{624};
t422 = ct{625};
t423 = ct{626};
t424 = ct{627};
t427 = ct{628};
t429 = ct{629};
t431 = ct{630};
t437 = ct{631};
t442 = ct{632};
t443 = ct{633};
t444 = ct{634};
t445 = ct{635};
t446 = ct{636};
t449 = ct{637};
t450 = ct{638};
t454 = ct{639};
t455 = ct{640};
t456 = ct{641};
t457 = ct{642};
t458 = ct{643};
t459 = ct{644};
t460 = ct{645};
t461 = ct{646};
t462 = ct{647};
t464 = ct{648};
t465 = ct{649};
t470 = ct{650};
t471 = ct{651};
t472 = ct{652};
t474 = ct{653};
t475 = ct{654};
t477 = ct{655};
t478 = ct{656};
t479 = ct{657};
t480 = ct{658};
t481 = ct{659};
t482 = ct{660};
t483 = ct{661};
t485 = ct{662};
t486 = ct{663};
t488 = ct{664};
t489 = ct{665};
t490 = ct{666};
t492 = ct{667};
t493 = ct{668};
t494 = ct{669};
t5 = ct{670};
t501 = ct{671};
t502 = ct{672};
t504 = ct{673};
t529 = ct{674};
t530 = ct{675};
t531 = ct{676};
t532 = ct{677};
t533 = ct{678};
t535 = ct{679};
t536 = ct{680};
t539 = ct{681};
t540 = ct{682};
t541 = ct{683};
t542 = ct{684};
t543 = ct{685};
t544 = ct{686};
t545 = ct{687};
t548 = ct{688};
t549 = ct{689};
t552 = ct{690};
t558 = ct{691};
t561 = ct{692};
t562 = ct{693};
t563 = ct{694};
t570 = ct{695};
t572 = ct{696};
t577 = ct{697};
t578 = ct{698};
t580 = ct{699};
t6 = ct{700};
t601 = ct{701};
t603 = ct{702};
t607 = ct{703};
t609 = ct{704};
t610 = ct{705};
t612 = ct{706};
t614 = ct{707};
t620 = ct{708};
t641 = ct{709};
t643 = ct{710};
t645 = ct{711};
t647 = ct{712};
t661 = ct{713};
t663 = ct{714};
t667 = ct{715};
t669 = ct{716};
t670 = ct{717};
t672 = ct{718};
t673 = ct{719};
t674 = ct{720};
t676 = ct{721};
t678 = ct{722};
t680 = ct{723};
t684 = ct{724};
t698 = ct{725};
t699 = ct{726};
t7 = ct{727};
t700 = ct{728};
t701 = ct{729};
t718 = ct{730};
t719 = ct{731};
t720 = ct{732};
t721 = ct{733};
t722 = ct{734};
t723 = ct{735};
t725 = ct{736};
t726 = ct{737};
t728 = ct{738};
t731 = ct{739};
t733 = ct{740};
t737 = ct{741};
t754 = ct{742};
t755 = ct{743};
t756 = ct{744};
t757 = ct{745};
t758 = ct{746};
t759 = ct{747};
t760 = ct{748};
t761 = ct{749};
t762 = ct{750};
t763 = ct{751};
t765 = ct{752};
t767 = ct{753};
t768 = ct{754};
t77 = ct{755};
t770 = ct{756};
t771 = ct{757};
t777 = ct{758};
t778 = ct{759};
t78 = ct{760};
t780 = ct{761};
t781 = ct{762};
t783 = ct{763};
t784 = ct{764};
t786 = ct{765};
t787 = ct{766};
t788 = ct{767};
t789 = ct{768};
t79 = ct{769};
t790 = ct{770};
t791 = ct{771};
t792 = ct{772};
t794 = ct{773};
t795 = ct{774};
t796 = ct{775};
t797 = ct{776};
t798 = ct{777};
t799 = ct{778};
t8 = ct{779};
t80 = ct{780};
t800 = ct{781};
t801 = ct{782};
t802 = ct{783};
t804 = ct{784};
t805 = ct{785};
t806 = ct{786};
t807 = ct{787};
t808 = ct{788};
t809 = ct{789};
t81 = ct{790};
t814 = ct{791};
t815 = ct{792};
t816 = ct{793};
t817 = ct{794};
t82 = ct{795};
t825 = ct{796};
t827 = ct{797};
t831 = ct{798};
t836 = ct{799};
t837 = ct{800};
t84 = ct{801};
t840 = ct{802};
t845 = ct{803};
t846 = ct{804};
t847 = ct{805};
t848 = ct{806};
t85 = ct{807};
t851 = ct{808};
t86 = ct{809};
t87 = ct{810};
t872 = ct{811};
t873 = ct{812};
t88 = ct{813};
t882 = ct{814};
t885 = ct{815};
t887 = ct{816};
t888 = ct{817};
t889 = ct{818};
t89 = ct{819};
t890 = ct{820};
t891 = ct{821};
t892 = ct{822};
t893 = ct{823};
t894 = ct{824};
t896 = ct{825};
t9 = ct{826};
t90 = ct{827};
t907 = ct{828};
t908 = ct{829};
t909 = ct{830};
t91 = ct{831};
t910 = ct{832};
t911 = ct{833};
t913 = ct{834};
t914 = ct{835};
t915 = ct{836};
t916 = ct{837};
t917 = ct{838};
t918 = ct{839};
t919 = ct{840};
t92 = ct{841};
t920 = ct{842};
t921 = ct{843};
t922 = ct{844};
t924 = ct{845};
t925 = ct{846};
t926 = ct{847};
t927 = ct{848};
t928 = ct{849};
t93 = ct{850};
t930 = ct{851};
t932 = ct{852};
t933 = ct{853};
t934 = ct{854};
t935 = ct{855};
t936 = ct{856};
t94 = ct{857};
t945 = ct{858};
t947 = ct{859};
t949 = ct{860};
t95 = ct{861};
t951 = ct{862};
t953 = ct{863};
t954 = ct{864};
t955 = ct{865};
t957 = ct{866};
t959 = ct{867};
t961 = ct{868};
t963 = ct{869};
t964 = ct{870};
t966 = ct{871};
t967 = ct{872};
t972 = ct{873};
t981 = ct{874};
t982 = ct{875};
t984 = ct{876};
t985 = ct{877};
t987 = ct{878};
t991 = ct{879};
t993 = ct{880};
t995 = ct{881};
t999 = ct{882};
th11_dot = ct{883};
th12_dot = ct{884};
th13_dot = ct{885};
th21_dot = ct{886};
th22_dot = ct{887};
th23_dot = ct{888};
th31_dot = ct{889};
th32_dot = ct{890};
th33_dot = ct{891};
th41_dot = ct{892};
th42_dot = ct{893};
th43_dot = ct{894};
zeta_dot = ct{895};
t2533 = t2420+t2504;
t2469 = t2375+t2443;
t2470 = t2377+t2442;
t2471 = t2376+t2446;
t2472 = t2379+t2447;
t2473 = t2396+t2452;
t2474 = t2397+t2453;
t2477 = t2398+t2458;
t2478 = t2400+t2457;
t2480 = t2403+t2460;
t2483 = -t2482;
t2486 = -t2484;
t2487 = -t2485;
t2490 = -t2488;
t2494 = -t2493;
t2499 = -t2497;
t2503 = -t2500;
t2506 = -t2502;
t2508 = -t2505;
t2511 = -t2507;
t2512 = -t2510;
t2518 = -t2517;
t2525 = t2390+t2491;
t2526 = t2389+t2492;
t2536 = t2426+t2501;
t2537 = t2422+t2509;
t2539 = t2428+t2513;
t2540 = t2429+t2515;
t2542 = t2431+t2516;
t2543 = t2427+t2519;
t2521 = t2386+t2483;
t2522 = t2384+t2490;
t2523 = t2392+t2486;
t2524 = t2393+t2487;
t2527 = t2391+t2494;
t2529 = t2412+t2499;
t2531 = t2414+t2506;
t2532 = t2419+t2503;
t2534 = t2413+t2508;
t2535 = t2410+t2511;
t2538 = t2417+t2512;
t2541 = t2425+t2518;
et1 = t437+t445+t446+t462+t754+t804+t805+t815+t817+t847+t924+t953+t954+t955+t964+t966+t967+t972+t1051+t1052+t1081+t1087+t1089+t1091+t1092+t1093+t1133+t1134+t1135+t1136+t1138+t1139+bx.*t577+bx.*t601+bx.*t609+bx.*t1053+bx_dot.*t530+bx_dot.*t549+bx_dot.*t1094+by.*t614+by.*t641+by.*t661+by.*t669+by.*t673+by.*t678+by.*t981+by.*t985+by.*t1105+by.*t1109-by_dot.*t78.*(9.0./2.0e+1)+by_dot.*t419+by_dot.*t806+by_dot.*t945-(p1x.*t162)./1.0e+1-p1x.*t265.*(7.0./2.0e+1)-(p1x.*t267)./1.0e+1-p1y.*t161.*(7.0./2.0e+1)-(p1y.*t163)./1.0e+1-(p1y.*t166)./1.0e+1+p1x.*t457+p1x.*t460+p1x.*t477-p1x_dot.*t77.*(7.0./2.0e+1)-(p1x_dot.*t79)./1.0e+1-p1x_dot.*t81.*(9.0./2.0e+1)-(p1y.*t254)./1.0e+1-p1x_dot.*t187.*(7.0./2.0e+1);
et2 = p1x.*t718+p1x.*t722+p1x.*t731+p1y.*t480-p1y_dot.*t80.*(7.0./2.0e+1)-(p1y_dot.*t82)./1.0e+1+p1x.*t801+p1x.*t848+p1x.*t882+p1x.*t887-(p1y_dot.*t217)./1.0e+1+p1x.*t909+p1x.*t930+p1x_dot.*t562+p1x.*t993+p1x.*t1006+p1x.*t1015+p1x.*t1061+p1x.*t1067+p1y_dot.*t424+p1x.*t1126+p1y.*t893+p1y.*t910+p1y.*t914+p1y.*t918+p1y_dot.*t501+p1y_dot.*t563+p1y.*t1027+p1y.*t1031+p1y.*t1076+p1x_dot.*t957-(bx.*t19.*t175)./5.0-(bx.*t84.*t161)./5.0-(bx.*t19.*t258)./5.0-(bx.*t180.*th11_dot)./5.0-(bx.*t380.*th11_dot)./5.0-p1y.*phi_dot.*t81.*(9.0./2.0e+1)-(p1x.*t19.*t162)./5.0-(p1y.*t19.*t163)./5.0-(p1y.*t19.*t166)./5.0-(p1x_dot.*t4.*t81)./5.0-(p1x_dot.*t19.*t79)./5.0;
et3 = p1y.*t19.*t254.*(-1.0./5.0)-(p1y_dot.*t19.*t82)./5.0-(p1y_dot.*t77.*t84)./5.0-(p1y.*t218.*th11_dot)./5.0-(p1y.*t222.*th11_dot)./5.0-(p1y.*t376.*th11_dot)./5.0-bx.*t17.*t31.*zeta_dot.*(9.0./2.0e+1)-(p1y.*phi_dot.*t4.*t81)./5.0-p1y.*t2.*t31.*zeta_dot.*(9.0./2.0e+1)-(bx.*t4.*t17.*t31.*zeta_dot)./5.0-(p1y.*t2.*t4.*t31.*zeta_dot)./5.0;
et4 = t2250.*(t1950.*(t798+t846+t888+t892+t907+t935+t1063+t1072+t2.*t366+t806.*zeta_dot+t945.*zeta_dot+phi_dot.*t17.*t242+psi_dot.*t18.*t529+(t16.*t19.*t164)./5.0-(t4.*t16.*t77.*th11_dot)./5.0)+t1948.*(t768+t794+t845+t936+t1047+t1049+t1065+t1071+t530.*zeta_dot+t1094.*zeta_dot+phi_dot.*t2.*t242-(psi_dot.*t18.*t180)./5.0+(t16.*t19.*t161)./5.0-(t17.*t84.*th11_dot)./5.0+t80.*t236.*th11_dot)+t1730.*t2058+t1823.*(t375+t465+t770+t796+t799+t3.*t352+t3.*t360+t242.*zeta_dot-(psi_dot.*t18.*t84)./5.0+(t16.*t19.*th11_dot)./5.0)-(t2.*t1571.*t2257)./2.0e+1-(t17.*t1571.*t2259)./2.0e+1).*1.0e+2;
et5 = t2251.*(t1730.*t1823+(t2.*t1571.*t1950)./2.0e+1-(t17.*t1571.*t1948)./2.0e+1).*(t2035+t2207+t2208-t2277-t2279+t2058.*(t209./5.0-t246)).*1.0e+4;
et6 = 1.0./(t1933+t1990.*(t1226-t1551)+t1998.*(t1266-t1559));
et7 = t2117.*(t489+t763+t846+t888+t892+t907+t1063+t1072-t777.*t1902+(t16.*t20.*t164)./5.0+(t77.*t85.*zeta_dot)./5.0+(psi_dot.*t18.*t20.*t78)./5.0-(t5.*t16.*t77.*th12_dot)./5.0-(t2.*t20.*t1084.*th12_dot)./1.0e+1)-t1907.*t2166-t1918.*(t374+t474+t486+t490+t765+t777.*t1601+(psi_dot.*t18.*t85)./5.0+(t20.*t1367.*th12_dot)./5.0-(t3.*t5.*t31.*th12_dot)./5.0-(t3.*t16.*t20.*zeta_dot)./5.0)+t2122.*(t845-t894+t936+t1065+t1071-t777.*t1896+t81.*zeta_dot.*(7.0./2.0e+1)+phi_dot.*t2.*t31.*(7.0./2.0e+1)+phi_dot.*t18.*t423+(t16.*t20.*t161)./5.0-(t80.*t85.*zeta_dot)./5.0-(psi_dot.*t18.*t20.*t81)./5.0+t16.*t80.*t145.*th12_dot+(t17.*t20.*t1084.*th12_dot)./1.0e+1)+(t2.*t1858.*t2317)./2.0e+1-(t17.*t1858.*t2325)./2.0e+1;
et8 = -2.0e+2;
et9 = ((-t1968.*t2317+t1967.*t2325-t2117.*(t456+t461+t479+t698+t873+t891+t908+t1062+t1066+t1075+(t20.*t1643)./5.0+(t102.*t777.*t1642)./2.0-(t5.*t1160.*th12_dot)./5.0-(t20.*t102.*t1070.*th12_dot)./1.0e+1)+t2122.*(t478+t701+t756+t759+t889+t911+t913+t919+t926+t1078+(t20.*t1645)./5.0+(t102.*t777.*t1644)./2.0+t145.*t1069.*th12_dot+(t20.*t102.*t1159.*th12_dot)./1.0e+1)+t1918.*(t475+t485+t494+t728+psi_dot.*t777.*t1074+t207.*t270.*t777+(t18.*t85.*zeta_dot)./5.0-(psi_dot.*t3.*t16.*t20)./5.0-(t5.*t16.*t18.*th12_dot)./5.0+(t16.*t20.*t270.*th12_dot)./1.0e+1)+(t16.*t1582.*t2166)./2.0e+1).*2.0e+2)./(t1933+t1990.*(t1226-t1551)+t1998.*(t1266-t1559));
et10 = t2344.*t2461.*(t1968.*t2117-t1967.*t2122+(t16.*t1582.*t1918)./2.0e+1).*-4.0e+4;
et11 = t2349.*(t2118.*(t489+t763+t846+t888+t892+t907+t1063+t1072+t778.*t1903+(t16.*t21.*t164)./5.0+(t77.*t86.*zeta_dot)./5.0+(psi_dot.*t18.*t21.*t78)./5.0-(t6.*t16.*t77.*th13_dot)./5.0-(t2.*t21.*t1165.*th13_dot)./1.0e+1)-t2127.*(t792+t890+t920+t925+t1013+t1079+t16.*t461+t778.*t1898+phi_dot.*t2.*t252-(t16.*t21.*t161)./5.0+(t80.*t86.*zeta_dot)./5.0+(psi_dot.*t18.*t21.*t81)./5.0-t16.*t80.*t146.*th13_dot-(t17.*t21.*t1165.*th13_dot)./1.0e+1)-t1904.*t2170+t1923.*(t273+t465+t770+t796+t799+t778.*t1614+t539.*zeta_dot-(psi_dot.*t18.*t86)./5.0-(t21.*t1326.*th13_dot)./5.0+t3.*t31.*t146.*th13_dot)-(t2.*t1851.*t2321)./2.0e+1+(t17.*t1851.*t2326)./2.0e+1).*-2.0e+2;
et12 = t2350.*t2468.*(t1904.*t1923-(t2.*t1851.*t2118)./2.0e+1+(t17.*t1851.*t2127)./2.0e+1).*-4.0e+4;
et13 = t2349.*(t2321.*(t217.*(7.0./2.0e+1)+t329+t427+t561-t1393-t1564)-t1960.*t2326+t2118.*(t456+t461+t479+t698+t873+t891+t908+t1062+t1066+t1075+(t21.*t1643)./5.0-(t102.*t778.*t1642)./2.0-(t6.*t1160.*th13_dot)./5.0+(t21.*t102.*t1070.*th13_dot)./1.0e+1)-t2127.*(t478+t701+t756+t759+t889+t911+t913+t919+t926+t1078+(t21.*t1645)./5.0-(t102.*t778.*t1644)./2.0+t146.*t1069.*th13_dot-(t21.*t102.*t1159.*th13_dot)./1.0e+1)+t1923.*(t450+t771+t795+t802+psi_dot.*t539+psi_dot.*t778.*t1074+t207.*t270.*t778-(t18.*t86.*zeta_dot)./5.0+t16.*t18.*t146.*th13_dot+(t16.*t21.*t270.*th13_dot)./1.0e+1)-(t16.*t1634.*t2170)./2.0e+1).*-2.0e+2;
et14 = t2350.*t2468.*(t2118.*(t217.*(7.0./2.0e+1)+t329+t427+t561-t1393-t1564)-t1960.*t2127+(t16.*t1634.*t1923)./2.0e+1).*-4.0e+4;
et15 = t445+t462+t754+t805+t814+t815+t816+t817+t831+t847+t896+t953+t964+t966+t972+t1051+t1081+t1083+t1086+t1093+t1133+t1135+t1138+t1139-bx.*t265.*(7.0./2.0e+1)+bx.*t603-bx.*t733+bx.*t1054+bx.*t1061+bx.*t1067-bx_dot.*t77.*(7.0./2.0e+1)-bx_dot.*t187.*(7.0./2.0e+1)+bx_dot.*t552+bx_dot.*t1096-by.*t161.*(7.0./2.0e+1)+by.*t643+by.*t663+by.*t670+by.*t987+by.*t1076+by.*t1106+by.*t1111-by_dot.*t78.*(9.0./2.0e+1)-by_dot.*t80.*(7.0./2.0e+1)+by_dot.*t420-by_dot.*t502+by_dot.*t947-(p2x.*t162)./1.0e+1-p2x.*t164.*(7.0./2.0e+1)-p2x.*t165.*(7.0./2.0e+1)-(p2x.*t267)./1.0e+1-(p2y.*t163)./1.0e+1-(p2y.*t166)./1.0e+1-p2y.*t176.*(7.0./2.0e+1)+p2x.*t477-(p2x_dot.*t79)./1.0e+1;
et16 = p2x_dot.*t81.*(-9.0./2.0e+1)-(p2y.*t254)./1.0e+1-p2y.*t257.*(7.0./2.0e+1)-p2x.*t578-p2x.*t610+p2y.*t442+p2x.*t719+p2x.*t723+p2x_dot.*t312-(p2y_dot.*t82)./1.0e+1+p2x.*t801-p2y_dot.*t177.*(7.0./2.0e+1)+p2x.*t887-(p2y_dot.*t217)./1.0e+1+p2x.*t909+p2x.*t915+p2x.*t922+p2x.*t928+p2x.*t930-p2y.*t674-p2y.*t680+p2x_dot.*t562+p2x_dot.*t572+p2x.*t995+p2y_dot.*t322+p2x.*t1016+p2y_dot.*t424+p2x.*t1127+p2y.*t914+p2y.*t918+p2y.*t932-p2y.*t982+p2y.*t1028+p2y.*t1033+p2y.*t1048+p2x_dot.*t959-(bx.*t22.*t175)./5.0-(bx.*t87.*t161)./5.0-(bx.*t22.*t258)./5.0+(bx_dot.*t7.*t81)./5.0-(bx.*t181.*th21_dot)./5.0+(bx.*t214.*th21_dot)./5.0;
et17 = (by.*t223.*th21_dot)./5.0+(by.*t377.*th21_dot)./5.0-p2y.*phi_dot.*t81.*(9.0./2.0e+1)-(p2x.*t22.*t162)./5.0-(p2y.*t22.*t163)./5.0-(p2y.*t22.*t166)./5.0-(p2x_dot.*t22.*t79)./5.0-(p2y.*t22.*t254)./5.0+p2x_dot.*t147.*t190+(p2y_dot.*t7.*t78)./5.0-(p2y_dot.*t22.*t82)./5.0-(p2y_dot.*t77.*t87)./5.0+(p2x.*t381.*th21_dot)./5.0-(p2y.*t219.*th21_dot)./5.0+(bx.*phi_dot.*t7.*t78)./5.0+(by.*phi_dot.*t7.*t81)./5.0+bx.*t147.*t308.*th21_dot-bx.*t17.*t31.*zeta_dot.*(9.0./2.0e+1)+p2y.*phi_dot.*t147.*t190-p2y.*t2.*t31.*zeta_dot.*(9.0./2.0e+1)+(by.*t2.*t7.*t31.*zeta_dot)./5.0+(p2x.*t7.*t17.*t31.*zeta_dot)./5.0;
et18 = t2254.*(t1952.*(t768+t794+t845+t890+t894+t1065+t1071+t1079+t532.*zeta_dot+t1096.*zeta_dot+phi_dot.*t2.*t243-(psi_dot.*t18.*t181)./5.0+(t16.*t22.*t161)./5.0-(t17.*t87.*th21_dot)./5.0+t80.*t237.*th21_dot)-t1731.*t2059+t1951.*(t798+t888+t892+t907+t917+t927+t935+t1014+t2.*t367+t807.*zeta_dot+t947.*zeta_dot+phi_dot.*t17.*t243+psi_dot.*t18.*t531+(t16.*t22.*t164)./5.0+t77.*t316.*th21_dot)+t1809.*(t375+t465+t474+t486+t799+t3.*t353+t3.*t361+t243.*zeta_dot-(psi_dot.*t18.*t87)./5.0+(t16.*t22.*th21_dot)./5.0)-(t2.*t1533.*t2253)./2.0e+1-(t17.*t1533.*t2258)./2.0e+1).*1.0e+2;
et19 = t2255.*(t1731.*t1809-(t2.*t1533.*t1951)./2.0e+1+(t17.*t1533.*t1952)./2.0e+1).*(t2012+t2209+t2212-t2275-t2278+t2059.*(t210./5.0-t247)).*-1.0e+4;
et20 = ((t2119.*(t489+t763+t888+t892+t907+t917+t927+t1014-t780.*t1902+(t16.*t23.*t164)./5.0+(t77.*t88.*zeta_dot)./5.0+(psi_dot.*t18.*t23.*t78)./5.0-(t8.*t16.*t77.*th22_dot)./5.0-(t2.*t23.*t1084.*th22_dot)./1.0e+1)+t2131.*(t471+t483+t845+t890+t894+t1065+t1071+t1079-t780.*t1896+(t16.*t23.*t161)./5.0-(t80.*t88.*zeta_dot)./5.0-(psi_dot.*t18.*t23.*t81)./5.0+t16.*t80.*t148.*th22_dot+(t17.*t23.*t1084.*th22_dot)./1.0e+1)-t1905.*t2167+t1915.*(t273+t465+t474+t486+t799-t780.*t1601+t541.*zeta_dot-(psi_dot.*t18.*t88)./5.0-(t23.*t1367.*th22_dot)./5.0+t3.*t31.*t148.*th22_dot)-(t2.*t1866.*t2315)./2.0e+1-(t17.*t1866.*t2327)./2.0e+1).*-2.0e+2)./(t1931+t1992.*(t1228-t1553)+t2011.*(t1271-t1560));
et21 = t2352.*t2463.*(t1905.*t1915-(t2.*t1866.*t2119)./2.0e+1+(t17.*t1866.*t2131)./2.0e+1).*-4.0e+4;
et22 = ((t1970.*t2315-t1969.*t2327+t2131.*(t444+t756+t759+t789+t913+t919+t926+t934+t1046+t1059+(t23.*t1645)./5.0+(t102.*t780.*t1644)./2.0+t148.*t1069.*th22_dot+(t23.*t102.*t1159.*th22_dot)./1.0e+1)-t2119.*(t260.*(7.0./2.0e+1)+t261.*(7.0./2.0e+1)+t479+t698+t757+t762-t873+t891+t908+t1075+(t23.*t1643)./5.0+(t102.*t780.*t1642)./2.0-t148.*t1160.*th22_dot-(t23.*t102.*t1070.*th22_dot)./1.0e+1)-t1915.*(t450+t475+t485+t802+psi_dot.*t541+psi_dot.*t780.*t1131+t270.*t272.*t780-(t18.*t88.*zeta_dot)./5.0+t16.*t18.*t148.*th22_dot-(t16.*t23.*t270.*th22_dot)./1.0e+1)+(t16.*t1599.*t2167)./2.0e+1).*2.0e+2)./(t1931+t1992.*(t1228-t1553)+t2011.*(t1271-t1560));
et23 = t2352.*t2463.*(t1970.*t2119+t1969.*t2131-(t16.*t1599.*t1915)./2.0e+1).*4.0e+4;
et24 = ((-t2120.*(t489+t763+t888+t892+t907+t917+t927+t1014+t781.*t1903+(t16.*t24.*t164)./5.0+(t77.*t89.*zeta_dot)./5.0+(psi_dot.*t18.*t24.*t78)./5.0-(t9.*t16.*t77.*th23_dot)./5.0-(t2.*t24.*t1165.*th23_dot)./1.0e+1)+t2128.*(t471+t483+t845+t890+t894+t1065+t1071+t1079-t781.*t1898+(t16.*t24.*t161)./5.0-(t80.*t89.*zeta_dot)./5.0-(psi_dot.*t18.*t24.*t81)./5.0+t16.*t80.*t149.*th23_dot+(t17.*t24.*t1165.*th23_dot)./1.0e+1)+t1899.*t2171-t1919.*(t273+t465+t474+t486+t799+t781.*t1614+t542.*zeta_dot-(psi_dot.*t18.*t89)./5.0-(t24.*t1326.*th23_dot)./5.0+t3.*t31.*t149.*th23_dot)+(t2.*t1847.*t2318)./2.0e+1+(t17.*t1847.*t2323)./2.0e+1).*2.0e+2)./(t1937-t2155+t1993.*(t1229-t1554));
et25 = t2346.*t2464.*(-t1899.*t1919+(t2.*t1847.*t2120)./2.0e+1+(t17.*t1847.*t2128)./2.0e+1).*4.0e+4;
et26 = (-t1962.*t2318+t1961.*t2323+t2120.*(t260.*(7.0./2.0e+1)+t261.*(7.0./2.0e+1)+t479+t698+t757+t762-t873+t891+t908+t1075+(t24.*t1643)./5.0-(t102.*t781.*t1642)./2.0-t149.*t1160.*th23_dot+(t24.*t102.*t1070.*th23_dot)./1.0e+1)+t1919.*(t450+t475+t485+t802+psi_dot.*t542+psi_dot.*t781.*t1074+t207.*t270.*t781-(t18.*t89.*zeta_dot)./5.0+t16.*t18.*t149.*th23_dot+(t16.*t24.*t270.*th23_dot)./1.0e+1)-t2128.*(t255.*(7.0./2.0e+1)+t258.*(7.0./2.0e+1)+t455+t458+t478+t701-t913-t919-t926-t934-(t24.*t1645)./5.0+(t102.*t781.*t1644)./2.0-(t9.*t1069.*th23_dot)./5.0+(t24.*t102.*t1159.*th23_dot)./1.0e+1)+(t16.*t1610.*t2171)./2.0e+1)./(t1937-t2155+t1993.*(t1229-t1554));
et27 = -2.0e+2;
et28 = t2239.*(t1945.*(t350+t359+t920+t925+t936+t1013+t1047+t1049+t17.*t368+t827.*zeta_dot+t961.*zeta_dot+psi_dot.*t18.*t405-(t16.*t25.*t161)./5.0+t80.*t317.*th31_dot-(phi_dot.*t2.*t10.*t31)./5.0)-t1664.*t2044+t1942.*(t343+t488+t888+t892+t907+t917+t927+t1014+t2.*t368+t808.*zeta_dot+t949.*zeta_dot+phi_dot.*t17.*t244+psi_dot.*t18.*t533+(t16.*t25.*t164)./5.0+t77.*t317.*th31_dot)+t1796.*(t465+t474+t486+t799+t3.*t354+t3.*t362-(t31.*zeta_dot)./4.0+t244.*zeta_dot-(psi_dot.*t18.*t90)./5.0+(t16.*t25.*th31_dot)./5.0)-(t2.*t1534.*t2248)./2.0e+1-(t17.*t1534.*t2252)./2.0e+1).*-1.0e+2;
et29 = t2240.*(-t1664.*t1796+(t2.*t1534.*t1942)./2.0e+1+(t17.*t1534.*t1945)./2.0e+1).*(t2005+t2201-t2203-t2272-t2274+t2044.*(t211./5.0-t248)).*1.0e+4;
et30 = t2353.*(t2112.*(t464+t797+t888+t892+t907+t917+t927+t1014-t783.*t1902+(t16.*t26.*t164)./5.0+(t77.*t91.*zeta_dot)./5.0+(psi_dot.*t18.*t26.*t78)./5.0-(t11.*t16.*t77.*th32_dot)./5.0-(t2.*t26.*t1084.*th32_dot)./1.0e+1)+t2134.*(t471+t483+t920+t925+t936+t1013+t1047+t1049+t783.*t1896-(t16.*t26.*t161)./5.0+(t80.*t91.*zeta_dot)./5.0+(psi_dot.*t18.*t26.*t81)./5.0-(t11.*t16.*t80.*th32_dot)./5.0-(t17.*t26.*t1084.*th32_dot)./1.0e+1)-t1900.*t2164-t1920.*(t273+t490+t765+t770+t796+t783.*t1601+(psi_dot.*t18.*t91)./5.0+(t26.*t1367.*th32_dot)./5.0-(t3.*t11.*t31.*th32_dot)./5.0-(t3.*t16.*t26.*zeta_dot)./5.0)-(t2.*t1867.*t2319)./2.0e+1+(t17.*t1867.*t2328)./2.0e+1).*-2.0e+2;
et31 = t2354.*t2465.*(t1900.*t1920+(t2.*t1867.*t2112)./2.0e+1+(t17.*t1867.*t2134)./2.0e+1).*4.0e+4;
et32 = ((t2113.*(t464+t797+t888+t892+t907+t917+t927+t1014+t784.*t1903+(t16.*t27.*t164)./5.0+(t77.*t92.*zeta_dot)./5.0+(psi_dot.*t18.*t27.*t78)./5.0-(t12.*t16.*t77.*th33_dot)./5.0-(t2.*t27.*t1165.*th33_dot)./1.0e+1)+t2123.*(t471+t483+t920+t925+t936+t1013+t1047+t1049+t784.*t1898-(t16.*t27.*t161)./5.0+(t80.*t92.*zeta_dot)./5.0+(psi_dot.*t18.*t27.*t81)./5.0-(t12.*t16.*t80.*th33_dot)./5.0-(t17.*t27.*t1165.*th33_dot)./1.0e+1)-t1897.*t2168+t1924.*(t374+t465+t474+t486+t799+t784.*t1614+t545.*zeta_dot-(psi_dot.*t18.*t92)./5.0-(t27.*t1326.*th33_dot)./5.0+t3.*t31.*t152.*th33_dot)+(t2.*t1859.*t2322)./2.0e+1-(t17.*t1859.*t2324)./2.0e+1).*-2.0e+2)./(t1941-t2149+t1984.*(t1231-t1556));
et33 = t2342.*t2466.*(-t1897.*t1924+(t2.*t1859.*t2113)./2.0e+1+(t17.*t1859.*t2123)./2.0e+1).*4.0e+4;
et34 = ((t1964.*t2322+t1963.*t2324+t2113.*(t260.*(7.0./2.0e+1)+t261.*(7.0./2.0e+1)+t479+t698+t757+t762-t873+t891+t908+t1075+(t27.*t1643)./5.0-(t102.*t784.*t1642)./2.0-t152.*t1160.*th33_dot+(t27.*t102.*t1070.*th33_dot)./1.0e+1)+t1924.*(t450+t475+t485+t802+psi_dot.*t545+psi_dot.*t784.*t1074+t207.*t270.*t784-(t18.*t92.*zeta_dot)./5.0+t16.*t18.*t152.*th33_dot+(t16.*t27.*t270.*th33_dot)./1.0e+1)-t2123.*(t255.*(7.0./2.0e+1)+t258.*(7.0./2.0e+1)+t455+t458+t478+t701-t913-t919-t926-t934-(t27.*t1645)./5.0+(t102.*t784.*t1644)./2.0-(t12.*t1069.*th33_dot)./5.0+(t27.*t102.*t1159.*th33_dot)./1.0e+1)+(t16.*t1611.*t2168)./2.0e+1).*-2.0e+2)./(t1941-t2149+t1984.*(t1231-t1556));
et35 = t2342.*t2466.*(t1964.*t2113-t1963.*t2123+(t16.*t1611.*t1924)./2.0e+1).*4.0e+4;
et36 = t437+t445+t446+t462+t804+t805+t815+t817+t847+t924+t954+t955+t966+t967+t1051+t1052+t1081+t1087+t1089+t1091+t1092+t1093+t1133+t1134+t1135+t1136+t1138+t1139+bx.*t371+bx.*t580+bx.*t607+bx.*t612+bx.*t1056-(bx_dot.*t81)./4.0+bx_dot.*t536+bx_dot.*t558+bx_dot.*t1098+by.*t470+by.*t481+by.*t620+by.*t647+by.*t667+by.*t672+by.*t676+by.*t684+by.*t984+by.*t991+by.*t1108+by.*t1115+by_dot.*t233+by_dot.*t422+by_dot.*t809+by_dot.*t951-(p4x.*t162)./1.0e+1-p4x.*t265.*(7.0./2.0e+1)-(p4x.*t267)./1.0e+1+p4x.*t341-p4y.*t161.*(7.0./2.0e+1)-(p4y.*t163)./1.0e+1-(p4y.*t166)./1.0e+1+p4x.*t457+p4x.*t460+p4x.*t477+p4x.*t492-p4x_dot.*t77.*(7.0./2.0e+1)-(p4x_dot.*t79)./1.0e+1-(p4y.*t254)./1.0e+1+p4y.*t351;
et37 = p4x_dot.*t187.*(-7.0./2.0e+1)+p4y.*t358+p4x_dot.*t241+p4x.*t721+p4x.*t725+p4y.*t480+p4x.*t737-(p4y_dot.*t78)./4.0-p4y_dot.*t80.*(7.0./2.0e+1)-(p4y_dot.*t82)./1.0e+1+p4x.*t851+p4x.*t885+p4x.*t887-(p4y_dot.*t217)./1.0e+1+p4x.*t909+p4x_dot.*t562+p4x.*t999+p4x.*t1012+p4x.*t1018+p4x.*t1061+p4x.*t1067+p4x.*t1129+p4y.*t893+p4y.*t910+p4y.*t914+p4y.*t918+p4y_dot.*t504+p4y_dot.*t563+p4y.*t1030+p4y.*t1037+p4y.*t1076+p4x_dot.*t963-(bx.*phi_dot.*t78)./4.0-(bx.*t28.*t175)./5.0-(bx.*t93.*t161)./5.0-(bx.*t28.*t258)./5.0-(bx.*t183.*th41_dot)./5.0-(bx.*t383.*th41_dot)./5.0-(p4x.*t28.*t162)./5.0-(p4y.*t28.*t163)./5.0-(p4y.*t28.*t166)./5.0-(p4x_dot.*t13.*t81)./5.0;
et38 = p4x_dot.*t28.*t79.*(-1.0./5.0)-(p4y.*t28.*t254)./5.0-(p4y_dot.*t28.*t82)./5.0-(p4y_dot.*t77.*t93)./5.0-(p4y.*t221.*th41_dot)./5.0-(p4y.*t225.*th41_dot)./5.0-(p4y.*t379.*th41_dot)./5.0-(p4y.*phi_dot.*t13.*t81)./5.0-(bx.*t13.*t17.*t31.*zeta_dot)./5.0-(p4y.*t2.*t13.*t31.*zeta_dot)./5.0;
et39 = t2244.*(t1810.*(t208+t474+t486+t490+t765+psi_dot.*t18.*t249-(t16.*t28.*th41_dot)./5.0-(t13.*t31.*zeta_dot)./5.0-(t3.*t13.*t31.*th41_dot)./5.0-(t3.*t16.*t28.*zeta_dot)./5.0)+t1701.*t2045+t1946.*(t350+t359+t890+t894+t920+t925+t1013+t1079+t17.*t369+t963.*zeta_dot+psi_dot.*t18.*t406-(t16.*t28.*t161)./5.0+t80.*t318.*th41_dot-(t13.*t81.*zeta_dot)./5.0-(phi_dot.*t2.*t13.*t31)./5.0)-t1943.*(t343+t488+t846+t888+t892+t907+t1063+t1072+t2.*t369+t809.*zeta_dot+t951.*zeta_dot+phi_dot.*t17.*t245+psi_dot.*t18.*t535+(t16.*t28.*t164)./5.0+t77.*t318.*th41_dot)+(t2.*t1572.*t2249)./2.0e+1+(t17.*t1572.*t2256)./2.0e+1).*-1.0e+2;
et40 = t2245.*(t1701.*t1810-(t2.*t1572.*t1943)./2.0e+1+(t17.*t1572.*t1946)./2.0e+1).*(t2013+t2202+t2204-t2273-t2276+t2045.*(t212./5.0-t249)).*-1.0e+4;
et41 = 1.0./(-t1932+t1985.*(t1232-t1557)+t2003.*(t1281-t1562));
et42 = (t2129.*(t471+t483+t890+t894+t920+t925+t1013+t1079+t786.*t1896-(t16.*t29.*t161)./5.0+(t80.*t94.*zeta_dot)./5.0+(psi_dot.*t18.*t29.*t81)./5.0-(t14.*t16.*t80.*th42_dot)./5.0-(t17.*t29.*t1084.*th42_dot)./1.0e+1)-t2114.*(t464+t797+t846+t888+t892+t907+t1063+t1072-t786.*t1902+(t16.*t29.*t164)./5.0+(t77.*t94.*zeta_dot)./5.0+(psi_dot.*t18.*t29.*t78)./5.0-(t14.*t16.*t77.*th42_dot)./5.0-(t2.*t29.*t1084.*th42_dot)./1.0e+1)+t1906.*t2165-t1916.*(t273+t474+t486+t490+t765+t786.*t1601+(psi_dot.*t18.*t94)./5.0+(t29.*t1367.*th42_dot)./5.0-(t3.*t14.*t31.*th42_dot)./5.0-(t3.*t16.*t29.*zeta_dot)./5.0)+(t2.*t1860.*t2316)./2.0e+1+(t17.*t1860.*t2329)./2.0e+1).*2.0e+2;
et43 = ((t1974.*t2316+t1973.*t2329-t2114.*(t456+t461+t479+t698+t873+t891+t908+t1062+t1066+t1075+(t29.*t1643)./5.0+(t102.*t786.*t1642)./2.0-(t14.*t1160.*th42_dot)./5.0-(t29.*t102.*t1070.*th42_dot)./1.0e+1)+t2129.*(t478+t701+t756+t759+t889+t911+t913+t919+t926+t1078+(t29.*t1645)./5.0+(t102.*t786.*t1644)./2.0+t154.*t1069.*th42_dot+(t29.*t102.*t1159.*th42_dot)./1.0e+1)-t1916.*(t475+t485+t494+t728+psi_dot.*t786.*t1074+t207.*t270.*t786+(t18.*t94.*zeta_dot)./5.0-(psi_dot.*t3.*t16.*t29)./5.0-(t14.*t16.*t18.*th42_dot)./5.0+(t16.*t29.*t270.*th42_dot)./1.0e+1)+(t16.*t1583.*t2165)./2.0e+1).*2.0e+2)./(-t1932+t1985.*(t1232-t1557)+t2003.*(t1281-t1562));
et44 = t2337.*(-t1974.*t2114+t1973.*t2129+(t16.*t1583.*t1916)./2.0e+1).*(t2173-t2191+t2293-t2306+t2356-t2373).*-4.0e+4;
et45 = (-t2132.*(t471+t483+t890+t894+t920+t925+t1013+t1079+t787.*t1898-(t16.*t30.*t161)./5.0+(t80.*t95.*zeta_dot)./5.0+(psi_dot.*t18.*t30.*t81)./5.0-(t15.*t16.*t80.*th43_dot)./5.0-(t17.*t30.*t1165.*th43_dot)./1.0e+1)+t2115.*(t464+t797+t846+t888+t892+t907+t1063+t1072+t787.*t1903+(t16.*t30.*t164)./5.0+(t77.*t95.*zeta_dot)./5.0+(psi_dot.*t18.*t30.*t78)./5.0-(t15.*t16.*t77.*th43_dot)./5.0-(t2.*t30.*t1165.*th43_dot)./1.0e+1)-t1901.*t2169+t1921.*(t273+t474+t486+t490+t765-t787.*t1614+(psi_dot.*t18.*t95)./5.0+(t30.*t1326.*th43_dot)./5.0-(t3.*t15.*t31.*th43_dot)./5.0-(t3.*t16.*t30.*zeta_dot)./5.0)+(t2.*t1868.*t2320)./2.0e+1+(t17.*t1868.*t2330)./2.0e+1)./(-t1938+t2157+t1986.*(t1233-t1558));
et46 = -2.0e+2;
et47 = ((t2320.*(t217.*(7.0./2.0e+1)+t329+t427+t561-t1408-t1570)+t1965.*t2330-t2115.*(t456+t461+t479+t698+t873+t891+t908+t1062+t1066+t1075+(t30.*t1643)./5.0-(t102.*t787.*t1642)./2.0-(t15.*t1160.*th43_dot)./5.0+(t30.*t102.*t1070.*th43_dot)./1.0e+1)+t2132.*(t478+t701+t756+t759+t889+t911+t913+t919+t926+t1078+(t30.*t1645)./5.0-(t102.*t787.*t1644)./2.0+t155.*t1069.*th43_dot-(t30.*t102.*t1159.*th43_dot)./1.0e+1)+t1921.*(t450+t771+t795+t802+psi_dot.*t548+psi_dot.*t787.*t1074+t207.*t270.*t787-(t18.*t95.*zeta_dot)./5.0+t16.*t18.*t155.*th43_dot+(t16.*t30.*t270.*th43_dot)./1.0e+1)+(t16.*t1635.*t2169)./2.0e+1).*2.0e+2)./(-t1938+t2157+t1986.*(t1233-t1558));
et48 = t2348.*t2467.*(-t2115.*(t217.*(7.0./2.0e+1)+t329+t427+t561-t1408-t1570)+t1965.*t2132+(t16.*t1635.*t1921)./2.0e+1).*-4.0e+4;
mt1 = [0.0,0.0,0.0,0.0,0.0,0.0,t2473,t2529,t2541,0.0,0.0,0.0,t2474,t2534,t2531,0.0,0.0,0.0,t2477,t2537,t2532,0.0,0.0,0.0,t2478,t2528,t2533,0.0,0.0,0.0,0.0,0.0,0.0,0.0,0.0,0.0,t2475,t2536,t2543,0.0,0.0,0.0,t2476,t2539,t2538,0.0,0.0,0.0,t2480,t2542,t2535,0.0,0.0,0.0,t2479,t2530,t2540,0.0,0.0,0.0,0.0,0.0,0.0,0.0,0.0,0.0,t2469,t2521,t2527,0.0,0.0,0.0,t2470,t2523,t2524,0.0,0.0,0.0,t2472,t2526,t2522,0.0,0.0,0.0,t2471,t2520,t2525,0.0,0.0,0.0,0.0,0.0,0.0,0.0,0.0,0.0,t2250.*(et1+et2+et3).*1.0e+2+t2251.*(t1950.*(t312+t319+t431+t530+t549+t572+t836+t1094)-t1948.*(t322+t328+t419+t570+t806+t825+t837+t945)).*(t2035+t2207+t2208-t2277-t2279+t2058.*(t209./5.0-t246)).*1.0e+4];
mt2 = [((t2092.*t2317-t2088.*t2325-t2122.*(t442+t454+t459+t472+t482+t790+t872+t932+t1048+t1058+t1060+t1064+t1315+t1716+t1759+t2072)+t2117.*(t443+t449+t758+t761+t788+t800+t915+t922+t928+t933+t1045+t1057+t1410+t1720+t1780+t2064)).*2.0e+2)./(t1933+t1990.*(t1226-t1551)+t1998.*(t1266-t1559))+t2344.*t2461.*(t2092.*t2117-t2088.*t2122).*4.0e+4,t2349.*(t2089.*t2326-t2102.*t2321+t2127.*(t442+t454+t459+t472+t482+t790+t872+t932+t1048+t1058+t1060+t1064+t1316+t1717+t1761+t2074)-t2118.*(t443+t449+t758+t761+t788+t800+t915+t922+t928+t933+t1045+t1057+t1411+t1665+t1781+t2076)).*-2.0e+2-t2350.*t2468.*(t2089.*t2127-t2102.*t2118).*4.0e+4,0.0,0.0,0.0];
mt3 = [t2254.*(et15+et16+et17).*1.0e+2+t2255.*(t1951.*(t319+t402+t431+t552+t836+t840-t959+(t7.*t81)./5.0)-t1952.*(t328+t420+t429+t563+t570+t807+t825+t947)).*(t2012+t2209+t2212-t2275-t2278+t2059.*(t210./5.0-t247)).*1.0e+4,((t2090.*t2327+t2107.*t2315-t2131.*(t454+t459+t472+t480+t482+t699+t872+t893+t910+t1060+t1064+t1076+t1318+t1718+t1765+t2073)-t2119.*(t477+t493+t700+t726+t758+t761+t887+t909+t915+t922+t928+t1077+t1452+t1703+t1736+t2077)).*2.0e+2)./(t1931+t1992.*(t1228-t1553)+t2011.*(t1271-t1560))-t2352.*t2463.*(t2090.*t2131-t2107.*t2119).*4.0e+4];
mt4 = [((t2091.*t2323-t2103.*t2318+t2128.*(t454+t459+t472+t480+t482+t699+t872+t893+t910+t1060+t1064+t1076+t1319+t1719+t1767+t2075)-t2120.*(t477+t493+t700+t726+t758+t761+t887+t909+t915+t922+t928+t1077+t1453+t1704+t1737+t2067)).*2.0e+2)./(t1937-t2155+t1993.*(t1229-t1554))+t2346.*t2464.*(t2091.*t2128-t2103.*t2120).*4.0e+4,0.0,0.0,0.0];
mt5 = [(t1939.*t2242-t1949.*t2234+t1966.*(t454+t459+t480+t645+t699+t767+t791+t872+t893+t910+t1060+t1064+t1076+t1208+t1212+t1320+t1769)-t1953.*(t449+t477+t700+t720+t758+t761+t800+t887+t909+t915+t922+t928+t1077+t1216+t1264+t1454+t1738))./(t2105+t1853.*(t211./5.0-t248)+t1966.*(t405-(t10.*t1159)./5.0))+(t2290.*t2435.*(t1949.*t1953-t1939.*t1966))./(t2105+t1853.*(t211./5.0-t248)+t1966.*(t405-(t10.*t1159)./5.0))];
mt6 = [t2353.*(t2084.*t2328+t2111.*t2319-t2112.*(t449+t477+t700+t758+t761+t800+t887+t909+t915+t922+t928+t1077+t1455+t1705+t1739+t2078)+t2134.*(t256.*(7.0./2.0e+1)+t454+t459-t472+t480-t482+t699+t872+t910-t932+t1060+t1064+t1771-t2055+(t11.*t1070.*th32_dot)./5.0-(t26.*t1637.*th32_dot)./5.0)).*2.0e+2-t2354.*t2465.*(t2084.*t2134-t2111.*t2112).*4.0e+4];
mt7 = [((t2085.*t2324+t2093.*t2322-t2113.*(t449+t477+t700+t758+t761+t800+t887+t909+t915+t922+t928+t1077+t1456+t1706+t1740+t2069)+t2123.*(t256.*(7.0./2.0e+1)+t454+t459-t472+t480-t482+t699+t872+t910-t932+t1060+t1064+t1773-t2062+(t12.*t1070.*th33_dot)./5.0-(t27.*t1636.*th33_dot)./5.0)).*2.0e+2)./(t1941-t2149+t1984.*(t1231-t1556))-t2342.*t2466.*(t2093.*t2113-t2085.*t2123).*4.0e+4,0.0,0.0,0.0,t2244.*(et36+et37+et38).*1.0e+2+t2245.*(t1943.*(t312+t319+t324+t536+t558+t572+t836+t1098)-t1946.*(t233+t322+t328+t422+t809+t825+t837+t951)).*(t2013+t2202+t2204-t2273-t2276+t2045.*(t212./5.0-t249)).*1.0e+4];
mt8 = [((t2086.*t2329+t2104.*t2316-t2129.*(t472+t480+t482+t699+t755+t760+t893+t910+t914+t918+t1039+t1076+t1365+t1699+t1793+t2056)+t2114.*(t457+t460+t477-t493+t700+t887+t909-t915-t922+t1073+t1077+t1707+t1742-t2070+phi_dot.*t78.*(7.0./2.0e+1)+t1436.*th42_dot)).*-2.0e+2)./(-t1932+t1985.*(t1232-t1557)+t2003.*(t1281-t1562))+t2337.*(t2086.*t2129-t2104.*t2114).*(t2173-t2191+t2293-t2306+t2356-t2373).*4.0e+4];
mt9 = [((t2087.*t2330+t2108.*t2320-t2132.*(t472+t480+t482+t699+t755+t760+t893+t910+t914+t918+t1039+t1076+t1366+t1700+t1795+t2063)+t2115.*(t457+t460+t477-t493+t700+t887+t909-t915-t922+t1073+t1077+t1743+t2071+phi_dot.*t78.*(7.0./2.0e+1)-(t15.*t1159.*th43_dot)./5.0-(t30.*t1629.*th43_dot)./5.0)).*-2.0e+2)./(-t1938+t2157+t1986.*(t1233-t1558))+t2348.*t2467.*(t2087.*t2132-t2108.*t2115).*4.0e+4,0.0,0.0,0.0,0.0,0.0,0.0,0.0,0.0,0.0,et4+et5,et6.*et7.*et8-t2344.*t2461.*(t1907.*t1918+(t2.*t1858.*t2117)./2.0e+1-(t17.*t1858.*t2122)./2.0e+1).*4.0e+4,et11+et12,0.0,0.0,0.0,et18+et19,et20+et21,et24+et25,0.0,0.0,0.0,et28+et29,et30+et31,et32+et33,0.0,0.0,0.0,et39+et40];
mt10 = [et41.*et42-t2337.*(t1906.*t1916-(t2.*t1860.*t2114)./2.0e+1+(t17.*t1860.*t2129)./2.0e+1).*(t2173-t2191+t2293-t2306+t2356-t2373).*4.0e+4,et45.*et46-t2348.*t2467.*(t1901.*t1921+(t2.*t1868.*t2115)./2.0e+1-(t17.*t1868.*t2132)./2.0e+1).*4.0e+4,0.0,0.0,0.0,0.0,0.0,0.0,0.0,0.0,0.0];
mt11 = [t2250.*(t1950.*(t456+t461+t479+t698+t873+t891+t908+t1062+t1066+t1075-(t19.*t161)./5.0+(t19.*t176)./5.0-(t84.*t175)./5.0+t162.*t246-(t4.*t80.*th11_dot)./5.0+t144.*t177.*th11_dot+t18.*t529.*zeta_dot)-t1948.*(t478+t701+t756+t759+t889+t911+t913+t919+t926+t1078-(t19.*t164)./5.0-(t19.*t165)./5.0+t163.*t246+t166.*t246+t77.*t144.*th11_dot+t144.*t187.*th11_dot+t18.*t403.*zeta_dot)-t1823.*(t475+t485+t494+t728+t18.*t246.*zeta_dot-(psi_dot.*t3.*t16.*t19)./5.0-(t4.*t16.*t18.*th11_dot)./5.0)+t1872.*t2259+t1876.*t2257-(t16.*t1150.*t2058)./2.0e+1).*1.0e+2-t2251.*(-t1872.*t1948+t1876.*t1950+(t16.*t1150.*t1823)./2.0e+1).*(t2035+t2207+t2208-t2277-t2279+t2058.*(t209./5.0-t246)).*1.0e+4];
mt12 = [et9+et10,et13+et14,0.0,0.0,0.0];
mt13 = [t2254.*(t1951.*(t479+t698+t757+t762+t891+t908+t916+t921+t1040+t1075-(t22.*t161)./5.0+(t22.*t176)./5.0-(t87.*t175)./5.0+t162.*t247-(t7.*t80.*th21_dot)./5.0+t147.*t177.*th21_dot+t18.*t531.*zeta_dot)-t1952.*(t444+t756+t759+t789+t913+t919+t926+t934+t1046+t1059-(t22.*t164)./5.0-(t22.*t165)./5.0+t163.*t247+t166.*t247+t77.*t147.*th21_dot+t147.*t187.*th21_dot+t18.*t404.*zeta_dot)-t1877.*t2253+t1873.*t2258+t1809.*(t450+t475+t485+t802+psi_dot.*t540+t18.*t237.*th21_dot-(t18.*t87.*zeta_dot)./5.0)-(t16.*t1171.*t2059)./2.0e+1).*1.0e+2+t2255.*(t1873.*t1952+t1877.*t1951-(t16.*t1171.*t1809)./2.0e+1).*(t2012+t2209+t2212-t2275-t2278+t2059.*(t210./5.0-t247)).*1.0e+4,et22+et23];
mt14 = [et26.*et27+t2346.*t2464.*(t1962.*t2120-t1961.*t2128+(t16.*t1610.*t1919)./2.0e+1).*4.0e+4,0.0,0.0,0.0];
mt15 = [t2239.*(t1942.*(t479+t698+t757+t762+t891+t908+t916+t921+t1040+t1075-(t25.*t161)./5.0+(t25.*t176)./5.0-(t90.*t175)./5.0+t162.*t248-(t10.*t80.*th31_dot)./5.0+t150.*t177.*th31_dot+t18.*t533.*zeta_dot)+t1945.*(t444+t756+t759+t789+t913+t919+t926+t934+t1046+t1059-(t25.*t164)./5.0-(t25.*t165)./5.0+t163.*t248+t166.*t248+t77.*t150.*th31_dot+t150.*t187.*th31_dot+t18.*t405.*zeta_dot)+t1874.*t2252-t1878.*t2248+t1796.*(t450+t475+t485+t802+psi_dot.*t543+t18.*t238.*th31_dot-(t18.*t90.*zeta_dot)./5.0)-(t16.*t1172.*t2044)./2.0e+1).*-1.0e+2-t2240.*(t1874.*t1945-t1878.*t1942+(t16.*t1172.*t1796)./2.0e+1).*(t2005+t2201-t2203-t2272-t2274+t2044.*(t211./5.0-t248)).*1.0e+4];
mt16 = [t2353.*(t1972.*t2319+t1971.*t2328+t2134.*(t444+t756+t759+t789+t913+t919+t926+t934+t1046+t1059+(t26.*t1645)./5.0+(t102.*t783.*t1644)./2.0+t151.*t1069.*th32_dot+(t26.*t102.*t1159.*th32_dot)./1.0e+1)+t2112.*(t260.*(7.0./2.0e+1)+t261.*(7.0./2.0e+1)+t479+t698+t757+t762-t873+t891+t908+t1075+(t26.*t1643)./5.0+(t102.*t783.*t1642)./2.0-t151.*t1160.*th32_dot-(t26.*t102.*t1070.*th32_dot)./1.0e+1)+t1920.*(t450+t475+t485+t802+psi_dot.*t544+psi_dot.*t783.*t1131+t270.*t272.*t783-(t18.*t91.*zeta_dot)./5.0+t16.*t18.*t151.*th32_dot-(t16.*t26.*t270.*th32_dot)./1.0e+1)-(t16.*t1600.*t2164)./2.0e+1).*-2.0e+2+t2354.*t2465.*(-t1972.*t2112+t1971.*t2134+(t16.*t1600.*t1920)./2.0e+1).*4.0e+4,et34+et35,0.0,0.0,0.0];
mt17 = [t2244.*(t1943.*(t456+t461+t479+t698+t873+t891+t908+t1062+t1066+t1075-(t28.*t161)./5.0+(t28.*t176)./5.0-(t93.*t175)./5.0+t162.*t249-(t13.*t80.*th41_dot)./5.0+t153.*t177.*th41_dot+t18.*t535.*zeta_dot)-t1946.*(t478+t701+t756+t759+t889+t911+t913+t919+t926+t1078-(t28.*t164)./5.0-(t28.*t165)./5.0+t163.*t249+t166.*t249+t77.*t153.*th41_dot+t153.*t187.*th41_dot+t18.*t406.*zeta_dot)+t1879.*t2249+t1875.*t2256-t1810.*(t475+t485+t494+t728+t18.*t318.*th41_dot+t18.*t249.*zeta_dot-(psi_dot.*t3.*t16.*t28)./5.0)-(t16.*t1151.*t2045)./2.0e+1).*1.0e+2-t2245.*(-t1875.*t1946+t1879.*t1943+(t16.*t1151.*t1810)./2.0e+1).*(t2013+t2202+t2204-t2273-t2276+t2045.*(t212./5.0-t249)).*1.0e+4,et43+et44];
mt18 = [et47+et48,0.0,0.0,0.0,0.0,0.0,0.0,0.0,0.0,0.0,t2473,t2529,t2541,0.0,0.0,0.0,0.0,0.0,0.0,0.0,0.0,0.0,0.0,0.0,0.0,0.0,0.0,0.0,0.0,0.0,0.0,0.0,0.0,0.0,0.0,0.0,0.0,0.0,0.0,0.0,t2475,t2536,t2543,0.0,0.0,0.0,0.0,0.0,0.0,0.0,0.0,0.0,0.0,0.0,0.0,0.0,0.0,0.0,0.0,0.0,0.0,0.0,0.0,0.0,0.0,0.0,0.0,0.0,0.0,0.0,t2469,t2521,t2527,0.0,0.0,0.0,0.0,0.0,0.0,0.0,0.0,0.0,0.0,0.0,0.0,0.0,0.0,0.0,0.0,0.0,0.0,0.0,0.0,0.0,0.0,0.0,0.0,0.0,0.0,0.0,0.0,0.0,0.0,0.0,0.0,0.0,t2474,t2534,t2531,0.0,0.0,0.0,0.0,0.0,0.0,0.0,0.0,0.0,0.0,0.0,0.0,0.0,0.0,0.0,0.0,0.0,0.0,0.0,0.0,0.0,0.0,0.0,0.0,0.0,0.0,0.0,t2476,t2539,t2538,0.0,0.0,0.0,0.0,0.0,0.0,0.0,0.0,0.0,0.0,0.0,0.0,0.0,0.0,0.0,0.0,0.0,0.0,0.0,0.0,0.0,0.0,0.0,0.0,0.0,0.0,0.0,t2470,t2523,t2524,0.0,0.0,0.0,0.0,0.0,0.0,0.0,0.0,0.0,0.0,0.0,0.0,0.0,0.0,0.0,0.0,0.0,0.0,0.0,0.0,0.0,0.0,0.0,0.0,0.0,0.0,0.0,0.0,0.0];
mt19 = [0.0,0.0,0.0,0.0,t2477,t2537,t2532,0.0,0.0,0.0,0.0,0.0,0.0,0.0,0.0,0.0,0.0,0.0,0.0,0.0,0.0,0.0,0.0,0.0,0.0,0.0,0.0,0.0,0.0,0.0,0.0,0.0,0.0,0.0,t2480,t2542,t2535,0.0,0.0,0.0,0.0,0.0,0.0,0.0,0.0,0.0,0.0,0.0,0.0,0.0,0.0,0.0,0.0,0.0,0.0,0.0,0.0,0.0,0.0,0.0,0.0,0.0,0.0,0.0,t2472,t2526,t2522,0.0,0.0,0.0,0.0,0.0,0.0,0.0,0.0,0.0,0.0,0.0,0.0,0.0,0.0,0.0,0.0,0.0,0.0,0.0,0.0,0.0,0.0,0.0,0.0,0.0,0.0,0.0,0.0,0.0,0.0,0.0,0.0,0.0,t2478,t2528,t2533,0.0,0.0,0.0,0.0,0.0,0.0,0.0,0.0,0.0,0.0,0.0,0.0,0.0,0.0,0.0,0.0,0.0,0.0,0.0,0.0,0.0,0.0,0.0,0.0,0.0,0.0,0.0,t2479,t2530,t2540,0.0,0.0,0.0,0.0,0.0,0.0,0.0,0.0,0.0,0.0,0.0,0.0,0.0,0.0,0.0,0.0,0.0,0.0,0.0,0.0,0.0,0.0,0.0,0.0,0.0,0.0,0.0,t2471,t2520,t2525,0.0,0.0,0.0];
S_dot = reshape([mt1,mt2,mt3,mt4,mt5,mt6,mt7,mt8,mt9,mt10,mt11,mt12,mt13,mt14,mt15,mt16,mt17,mt18,mt19],30,18);
end
